simulink model "generic_IVS"  (R2024a)
settings: Solver=FixedStepDiscrete  StartTime=0.0  StopTime=inf  FixedStep=0.001  RelTol=1e-3
undefined symbols (not defined in the file): do_waypoints_tail_shifted_2, pathXY, route1_waypoint, route1_waypoint_raw, route2_waypoint, route2_waypoint_raw, route3_waypoint, route3_waypoint_raw, waypoints2
libraries: CarMaker4SL x431, slpidlib x19, dspsigops x3, simulink x1
(part 3 of 15)

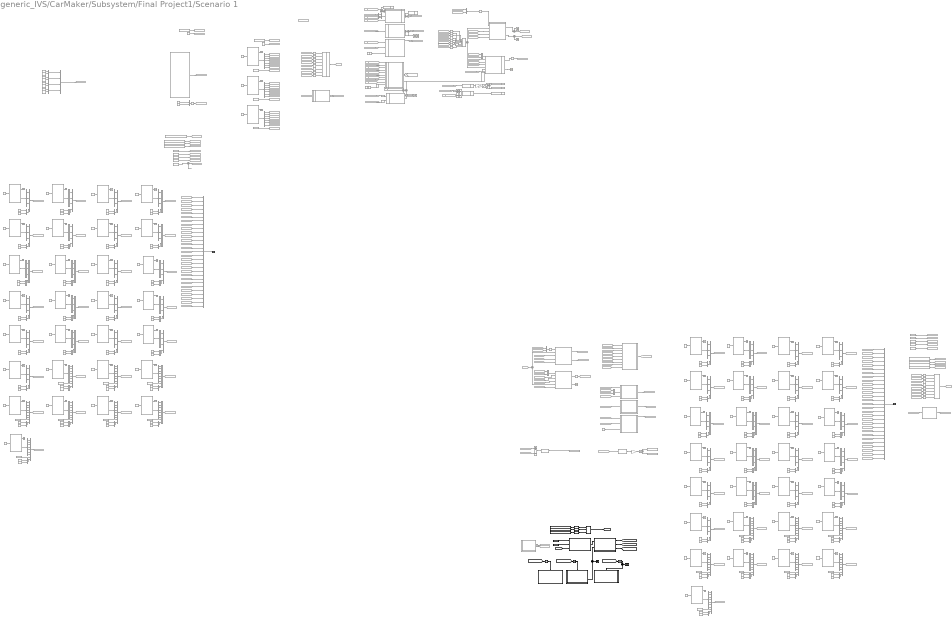
== system generic_IVS/CarMaker/Subsystem/Final Project1/Scenario 1 ==
  note: Average Filter
  note: Do Not Modify !!
  note: Traffic Size
      | Length: 4.47
      | Width: 1.97
      | Height: 1.12
  note: Modify !!
  note: Traffic Size
      | Length: 4.47
      | Width: 1.97
      | Height: 1.12
  note: Traffic Size
      | Length: 4.47
      | Width: 1.97
      | Height: 1.12
  note: *** Final Project ***
      |
      | Scenario:
      | Input:
      | Output:
      | 제어기 10ms / 다익스트라 1s
  note: Do Not Modify !!
  note: Traffic Size
      | Length: 4.47
      | Width: 1.97
      | Height: 1.12
  note: Traffic Size
      | Length: 4.47
      | Width: 1.97
      | Height: 1.12
  note: Traffic Size
      | Length: 4.47
      | Width: 1.97
      | Height: 1.12
  note: Traffic Size
      | Length: 4.47
      | Width: 1.97
      | Height: 1.12
  note: Traffic Size
      | Length: 4.47
      | Width: 1.97
      | Height: 1.12
  note: Traffic Size
      | Length: 4.47
      | Width: 1.97
      | Height: 1.12
  note: Traffic Size
      | Length: 4.47
      | Width: 1.97
      | Height: 1.12
  note: Traffic Size
      | Length: 4.47
      | Width: 1.97
      | Height: 1.12
  note: Traffic Size
      | Length: 4.47
      | Width: 1.97
      | Height: 1.12
  note: Traffic Size
      | Length: 4.47
      | Width: 1.97
      | Height: 1.12
  note: Traffic Size
      | Length: 4.47
      | Width: 1.97
      | Height: 1.12
  note: Traffic Size
      | Length: 4.47
      | Width: 1.97
      | Height: 1.12
  note: Traffic Size
      | Length: 4.47
      | Width: 1.97
      | Height: 1.12
  note: Traffic Size
      | Length: 4.47
      | Width: 1.97
      | Height: 1.12
  note: Traffic Size
      | Length: 4.47
      | Width: 1.97
      | Height: 1.12
  note: Traffic Size
      | Length: 4.47
      | Width: 1.97
      | Height: 1.12
  note: Traffic Size
      | Length: 4.47
      | Width: 1.97
      | Height: 1.12
  note: Traffic Size
      | Length: 4.47
      | Width: 1.97
      | Height: 1.12
  note: Traffic Size
      | Length: 4.47
      | Width: 1.97
      | Height: 1.12
  note: Traffic Size
      | Length: 4.47
      | Width: 1.97
      | Height: 1.12
  note: Traffic Size
      | Length: 4.47
      | Width: 1.97
      | Height: 1.12
  note: Traffic Size
      | Length: 4.47
      | Width: 1.97
      | Height: 1.12
  note: Traffic Size
      | Length: 4.47
      | Width: 1.97
      | Height: 1.12
  note: Traffic Size
      | Length: 4.47
      | Width: 1.97
      | Height: 1.12
  note: Traffic Size
      | Length: 4.47
      | Width: 1.97
      | Height: 1.12
  note: Traffic Size
      | Length: 4.47
      | Width: 1.97
      | Height: 1.12
  note: Traffic Size
      | Length: 4.47
      | Width: 1.97
      | Height: 1.12
  note: Traffic Size
      | Length: 4.47
      | Width: 1.97
      | Height: 1.12
  note: Traffic Size
      | Length: 4.47
      | Width: 1.97
      | Height: 1.12
  note: Traffic Size
      | Length: 4.47
      | Width: 1.97
      | Height: 1.12
  note: Traffic Size
      | Length: 4.47
      | Width: 1.97
      | Height: 1.12
  note: Traffic Size
      | Length: 4.47
      | Width: 1.97
      | Height: 1.12
  note: Traffic Size
      | Length: 4.47
      | Width: 1.97
      | Height: 1.12
  note: *** Final Project ***
      |
      | Scenario:
      | Input:
      | Output:
      | 제어기 10ms / 다익스트라 1s
  note: Traffic Size
      | Length: 4.47
      | Width: 1.97
      | Height: 1.12
  note: Average Filter
  note: Traffic Size
      | Length: 4.47
      | Width: 1.97
      | Height: 1.12
  note: Traffic Size
      | Length: 4.47
      | Width: 1.97
      | Height: 1.12
  note: Traffic Size
      | Length: 4.47
      | Width: 1.97
      | Height: 1.12
  note: Traffic Size
      | Length: 4.47
      | Width: 1.97
      | Height: 1.12
  note: Traffic Size
      | Length: 4.47
      | Width: 1.97
      | Height: 1.12
  note: Traffic Size
      | Length: 4.47
      | Width: 1.97
      | Height: 1.12
  note: Traffic Size
      | Length: 4.47
      | Width: 1.97
      | Height: 1.12
  note: Traffic Size
      | Length: 4.47
      | Width: 1.97
      | Height: 1.12
  note: Traffic Size
      | Length: 4.47
      | Width: 1.97
      | Height: 1.12
  note: Traffic Size
      | Length: 4.47
      | Width: 1.97
      | Height: 1.12
  note: Traffic Size
      | Length: 4.47
      | Width: 1.97
      | Height: 1.12
  note: Traffic Size
      | Length: 4.47
      | Width: 1.97
      | Height: 1.12
  note: Traffic Size
      | Length: 4.47
      | Width: 1.97
      | Height: 1.12
  note: Traffic Size
      | Length: 4.47
      | Width: 1.97
      | Height: 1.12
  note: Traffic Size
      | Length: 4.47
      | Width: 1.97
      | Height: 1.12
  note: Traffic Size
      | Length: 4.47
      | Width: 1.97
      | Height: 1.12
  note: Modify !!
  note: Traffic Size
      | Length: 4.47
      | Width: 1.97
      | Height: 1.12
  note: Traffic Size
      | Length: 4.47
      | Width: 1.97
      | Height: 1.12
  note: Traffic Size
      | Length: 4.47
      | Width: 1.97
      | Height: 1.12
  note: Traffic Size
      | Length: 4.47
      | Width: 1.97
      | Height: 1.12
  note: Traffic Size
      | Length: 4.47
      | Width: 1.97
      | Height: 1.12
  note: Traffic Size
      | Length: 4.47
      | Width: 1.97
      | Height: 1.12
  note: Traffic Size
      | Length: 4.47
      | Width: 1.97
      | Height: 1.12
  note: Traffic Size
      | Length: 4.47
      | Width: 1.97
      | Height: 1.12
  note: Do Not Modify !!
  note: Average Filter
  note: Modify !!
  Add : Sum  Commented=on  Inputs=+-
  Add1 : Sum  Commented=on  Inputs=+-
  Add2 : Sum  Commented=on  Inputs=+-
  Bus Selector{,1..2,20..21,23..27,31,42..43,45..49,54} (19 alike) : BusSelector  Commented=on  OutputSignals=t_0 x,t_0 y,v_0 x,v_0 y,a_0 x,a_0 y,r_zyx z
  Bus Selector{3..19,22,28..30,32..41,44,50..53,55..60} (42 alike) : BusSelector  Commented=on  OutputSignals=t_0 x,t_0 y,r_zyx z
  Chart : Stateflow chart  Commented=on  TreatAsAtomicUnit=on
  Constant : Constant  Commented=on  Value=80
  Constant1 : Constant  Commented=on  Value=0
  Constant10 : Constant  Commented=on  Value=2.48
  Constant100 : Constant  Commented=on  Value=47.5
  Constant101 : Constant  Commented=on  Value=-45
  Constant102 : Constant  Commented=on  Value=5.5
  Constant103 : Constant  Commented=on  Value=-45
  Constant104 : Constant  Commented=on  Value=47.5
  Constant105 : Constant  Commented=on  Value=-4
  Constant106 : Constant  Commented=on  Value=pathXY
  Constant107 : Constant  Commented=on  Value=pathXY
  Constant{2,7,11,108,168,202} (6 alike) : Constant  Commented=on
  Constant109 : Constant  Commented=on  Value=5
  Constant{13,16,19,21..22,26,29,32,35,39,42,46,48,52,55..56,59,61,65,69,72,74,79,82,85,87..88,92,96,110,113,116,118..119,123,126,129,132,136,139,143,145,149,152..153,156,159,163,167,171,173,178,182,185,187..188,193,197} (58 alike) : Constant  Commented=on  Value=4.47
  Constant{14,17,23..24,27,30,33,36..37,40,43,49..50,53,57,62..63,66..67,70,75..76,80,83,89..90,93..94,97,111,114,120..121,124,127,130,133..134,137,140,146..147,150,154,160..161,164..165,169,174..175,180,183,189,191,194..195,198} (58 alike) : Constant  Commented=on  Value=1.97
  Constant112 : Constant  Commented=on  Value=7
  Constant115 : Constant  Commented=on  Value=8
  Constant117 : Constant  Commented=on  Value=4
  Constant12 : Constant  Commented=on  Value=5
  Constant122 : Constant  Commented=on  Value=10
  Constant125 : Constant  Commented=on  Value=11
  Constant128 : Constant  Commented=on  Value=12
  Constant131 : Constant  Commented=on  Value=9
  Constant135 : Constant  Commented=on  Value=14
  Constant138 : Constant  Commented=on  Value=15
  Constant141 : Constant  Commented=on  Value=2
  Constant142 : Constant  Commented=on  Value=16
  Constant144 : Constant  Commented=on  Value=13
  Constant148 : Constant  Commented=on  Value=18
  Constant15 : Constant  Commented=on  Value=7
  Constant151 : Constant  Commented=on  Value=19
  Constant155 : Constant  Commented=on  Value=6
  Constant157 : Constant  Commented=on  Value=route1_waypoint_raw
  Constant158 : Constant  Commented=on  Value=17
  Constant162 : Constant  Commented=on  Value=21
  Constant166 : Constant  Commented=on  Value=22
  Constant170 : Constant  Commented=on  Value=23
  Constant172 : Constant  Commented=on  Value=20
  Constant176 : Constant  Commented=on  Value=3
  Constant177 : Constant  Commented=on  Value=25
  Constant179 : Constant  Commented=on  Value=route2_waypoint_raw
  Constant18 : Constant  Commented=on  Value=8
  Constant181 : Constant  Commented=on  Value=26
  Constant184 : Constant  Commented=on  Value=27
  Constant186 : Constant  Commented=on  Value=24
  Constant190 : Constant  Commented=on  Value=route3_waypoint_raw
  Constant192 : Constant  Commented=on  Value=0
  Constant196 : Constant  Commented=on  Value=28
  Constant199 : Constant  Value=route1_waypoint  SampleTime=-1
  Constant20 : Constant  Commented=on  Value=4
  Constant200 : Constant  Value=route2_waypoint  SampleTime=-1
  Constant201 : Constant  Value=route3_waypoint  SampleTime=-1
  Constant25 : Constant  Commented=on  Value=10
  Constant28 : Constant  Commented=on  Value=11
  Constant3 : Constant  Commented=on  Value=2
  Constant31 : Constant  Commented=on  Value=12
  Constant34 : Constant  Commented=on  Value=9
  Constant38 : Constant  Commented=on  Value=14
  Constant4 : Constant  Commented=on  Value=80
  Constant41 : Constant  Commented=on  Value=15
  Constant44 : Constant  Commented=on  Value=2
  Constant45 : Constant  Commented=on  Value=16
  Constant47 : Constant  Commented=on  Value=13
  Constant5 : Constant  Commented=on  Value=11.5
  Constant51 : Constant  Commented=on  Value=18
  Constant54 : Constant  Commented=on  Value=19
  Constant58 : Constant  Commented=on  Value=6
  Constant6 : Constant  Commented=on  Value=route1_waypoint_raw
  Constant60 : Constant  Commented=on  Value=17
  Constant64 : Constant  Commented=on  Value=21
  Constant68 : Constant  Commented=on  Value=22
  Constant71 : Constant  Commented=on  Value=23
  Constant73 : Constant  Commented=on  Value=20
  Constant77 : Constant  Commented=on  Value=3
  Constant78 : Constant  Commented=on  Value=25
  Constant8 : Constant  Commented=on  Value=route2_waypoint_raw
  Constant81 : Constant  Commented=on  Value=26
  Constant84 : Constant  Commented=on  Value=27
  Constant86 : Constant  Commented=on  Value=24
  Constant9 : Constant  Commented=on  Value=route3_waypoint_raw
  Constant91 : Constant  Commented=on  Value=0
  Constant95 : Constant  Commented=on  Value=28
  Constant98 : Constant  Commented=on  Value=5.5
  Constant99 : Constant  Commented=on  Value=-4
  Display : Display  Commented=on
  Display1 : Display  Commented=on
  Enabled Subsystem : Subsystem  TreatAsAtomicUnit=on
  Enabled Subsystem1 : Subsystem  TreatAsAtomicUnit=on
  Enabled Subsystem2 : Subsystem  TreatAsAtomicUnit=on
  From : From  Commented=on  GotoTag=Traffic_Info_00
  From1 : From  Commented=on  GotoTag=Traffic_Info_01
  From10 : From  Commented=on  GotoTag=Traffic_Info_10
  From100 : From  Commented=on  GotoTag=LateralError
  From101 : From  Commented=on  GotoTag=Global_Waypoints1
  From{2,35,73..74,102,136..137,163} (8 alike) : From  Commented=on  GotoTag=Global_Waypoints2
  From103 : From  Commented=on  GotoTag=Global_Waypoints3
  From{4,28,37,63,77,104,126,133,140,152,155,166} (12 alike) : From  Commented=on  GotoTag=Ego_Global_X
  From{5,29,38,64,78,105,127,141,143,153,156,167} (12 alike) : From  Commented=on  GotoTag=Ego_Gloabl_Y
  From{39,56,69,106,132} (5 alike) : From  Commented=on  GotoTag=Traffic_Info_27
  From107 : From  Commented=on  GotoTag=Traffic_Info_01
  From{40,70,72,108,134} (5 alike) : From  Commented=on  GotoTag=Traffic_Info_28
  From109 : From  Commented=on  GotoTag=Traffic_Info_03
  From11 : From  Commented=on  GotoTag=Traffic_Info_11
  From110 : From  Commented=on  GotoTag=Traffic_Info_04
  From111 : From  Commented=on  GotoTag=Traffic_Info_05
  From112 : From  Commented=on  GotoTag=Traffic_Info_06
  From113 : From  Commented=on  GotoTag=Traffic_Info_07
  From114 : From  Commented=on  GotoTag=Traffic_Info_08
  From115 : From  Commented=on  GotoTag=Traffic_Info_09
  From{76,116,139,165} (4 alike) : From  Commented=on  GotoTag=onRoad_Traffic
  From{8,54,71,79,98,117,135,142,157,168..169} (11 alike) : From  Commented=on  GotoTag=Ego_Velocity
  From{55,82,118,146,158,172} (6 alike) : From  Commented=on  GotoTag=Target_speed2
  From119 : From  Commented=on  GotoTag=Trajectory
  From12 : From  Commented=on  GotoTag=Traffic_Info_12
  From{22,48,58,91,120} (5 alike) : From  Commented=on  GotoTag=Traffic_Info_21
  From{23,49,59,92,121} (5 alike) : From  Commented=on  GotoTag=Traffic_Info_22
  From{3,65,81,122,128,145,154,171} (8 alike) : From  Commented=on  GotoTag=Ego_Yaw
  From{24,50,60,93,123} (5 alike) : From  Commented=on  GotoTag=Traffic_Info_23
  From{25,51,61,94,124} (5 alike) : From  Commented=on  GotoTag=Traffic_Info_24
  From{26,52,62,95,125} (5 alike) : From  Commented=on  GotoTag=Traffic_Info_25
  From129 : From  Commented=on  GotoTag=ego_lane_idx
  From13 : From  Commented=on  GotoTag=Traffic_Info_13
  From130 : From  Commented=on  GotoTag=traffic_lane_idx
  From{27,53,68,96,131} (5 alike) : From  Commented=on  GotoTag=Traffic_Info_26
  From138 : From  Commented=on  GotoTag=s_reference
  From14 : From  Commented=on  GotoTag=Traffic_Info_14
  From144 : From  Commented=on  GotoTag=Ego_Accel
  From147 : From  Commented=on  GotoTag=Local_Points
  From15 : From  Commented=on  GotoTag=Traffic_Info_15
  From159 : From  Commented=on  GotoTag=Trajectory
  From16 : From  Commented=on  GotoTag=Traffic_Info_16
  From160 : From  Commented=on  GotoTag=Local_Points
  From161 : From  Commented=on  GotoTag=traffic_lane_idx
  From162 : From  Commented=on  GotoTag=Coefficients
  From164 : From  Commented=on  GotoTag=s_reference
  From17 : From  Commented=on  GotoTag=Traffic_Info_17
  From170 : From  Commented=on  GotoTag=Ego_Accel
  From173 : From  Commented=on  GotoTag=LateralError
  From18 : From  Commented=on  GotoTag=Traffic_Info_18
  From19 : From  Commented=on  GotoTag=Traffic_Info_19
  From20 : From  Commented=on  GotoTag=Traffic_Info_02
  From21 : From  Commented=on  GotoTag=Traffic_Info_20
  From30 : From  Commented=on  GotoTag=Traffic_Info_10
  From31 : From  Commented=on  GotoTag=Traffic_Info_11
  From32 : From  Commented=on  GotoTag=Traffic_Info_12
  From33 : From  Commented=on  GotoTag=Traffic_Info_13
  From34 : From  Commented=on  GotoTag=Global_Waypoints1
  From36 : From  Commented=on  GotoTag=Global_Waypoints3
  From41 : From  Commented=on  GotoTag=Traffic_Info_03
  From42 : From  Commented=on  GotoTag=Traffic_Info_04
  From43 : From  Commented=on  GotoTag=Traffic_Info_05
  From44 : From  Commented=on  GotoTag=Traffic_Info_06
  From45 : From  Commented=on  GotoTag=Traffic_Info_07
  From46 : From  Commented=on  GotoTag=Traffic_Info_08
  From47 : From  Commented=on  GotoTag=Traffic_Info_09
  From57 : From  Commented=on  GotoTag=Trajectory
  From6 : From  Commented=on  GotoTag=Local_Points
  From66 : From  Commented=on  GotoTag=ego_lane_idx
  From67 : From  Commented=on  GotoTag=traffic_lane_idx
  From7 : From  Commented=on  GotoTag=Coefficients
  From75 : From  Commented=on  GotoTag=s_reference
  From80 : From  Commented=on  GotoTag=Ego_Accel
  From83 : From  Commented=on  GotoTag=Traffic_Info_14
  From84 : From  Commented=on  GotoTag=Traffic_Info_15
  From85 : From  Commented=on  GotoTag=Traffic_Info_16
  From86 : From  Commented=on  GotoTag=Traffic_Info_17
  From87 : From  Commented=on  GotoTag=Traffic_Info_18
  From88 : From  Commented=on  GotoTag=Traffic_Info_19
  From89 : From  Commented=on  GotoTag=Traffic_Info_02
  From9 : From  Commented=on  GotoTag=LateralError
  From90 : From  Commented=on  GotoTag=Traffic_Info_20
  From97 : From  Commented=on  GotoTag=Coefficients
  From99 : From  Commented=on  GotoTag=Traffic_Info_00
  Function-Call Split : FunctionCallSplit  Commented=on  IconShape=distinctive  NumOutputPorts=2  OutputPortLayout=default
  Gain : Gain  Commented=on  Gain=pi/180
  Gain1 : Gain  Commented=on  Gain=pi/180
  Gain2 : Gain  Commented=on  Gain=pi/180
  Goto : Goto  Commented=on  GotoTag=onRoad_Traffic
  Goto1 : Goto  Commented=on  GotoTag=CrossTrackError
  Goto10 : Goto  Commented=on  GotoTag=Traffic00_Yaw
  Goto100 : Goto  Commented=on  GotoTag=Traffic_Info_19
  Goto101 : Goto  Commented=on  GotoTag=Traffic_Info_17
  Goto102 : Goto  Commented=on  GotoTag=Traffic_Info_06
  Goto103 : Goto  Commented=on  GotoTag=Traffic_Info_02
  Goto104 : Goto  Commented=on  GotoTag=Traffic_Info_21
  Goto105 : Goto  Commented=on  GotoTag=Traffic_Info_22
  Goto106 : Goto  Commented=on  GotoTag=Traffic_Info_20
  Goto107 : Goto  Commented=on  GotoTag=Traffic_Info_23
  Goto108 : Goto  Commented=on  GotoTag=Traffic_Info_25
  Goto109 : Goto  Commented=on  GotoTag=Traffic_Info_26
  Goto11 : Goto  Commented=on  GotoTag=Traffic01_Yaw
  Goto110 : Goto  Commented=on  GotoTag=Traffic_Info_24
  Goto111 : Goto  Commented=on  GotoTag=Traffic_Info_27
  Goto112 : Goto  Commented=on  GotoTag=Traffic_Info_00
  Goto113 : Goto  Commented=on  GotoTag=Traffic_Info_03
  Goto114 : Goto  Commented=on  GotoTag=Traffic_Info_28
  Goto115 : Goto  Commented=on  GotoTag=Traffic_Info_05
  Goto116 : Goto  Commented=on  GotoTag=Traffic_Info_07
  Goto117 : Goto  Commented=on  GotoTag=Traffic_Info_04
  Goto118 : Goto  Commented=on  GotoTag=Traffic_Info_08
  Goto119 : Goto  Commented=on  GotoTag=Traffic_Info_10
  Goto12 : Goto  Commented=on  GotoTag=Traffic01_YawRate
  Goto120 : Goto  Commented=on  GotoTag=Traffic_Info_11
  Goto121 : Goto  Commented=on  GotoTag=Global_Waypoints4
  Goto122 : Goto  Commented=on  GotoTag=s_reference
  Goto123 : Goto  Commented=on  GotoTag=Trajectory
  Goto124 : Goto  Commented=on  GotoTag=Ego_Accel
  Goto125 : Goto  Commented=on  GotoTag=do_Logic
  Goto126 : Goto  Commented=on  GotoTag=do_Logic_
  Goto13 : Goto  Commented=on  GotoTag=Traffic01_Global_X
  Goto131 : Goto  Commented=on  GotoTag=Local_Points
  Goto132 : Goto  Commented=on  GotoTag=Coefficients
  Goto133 : Goto  Commented=on  GotoTag=LateralError
  Goto134 : Goto  Commented=on  GotoTag=s_reference
  Goto135 : Goto  Commented=on  GotoTag=Trajectory
  Goto14 : Goto  Commented=on  GotoTag=Traffic01_Global_Y
  Goto15 : Goto  Commented=on  GotoTag=Traffic01_Vx
  Goto16 : Goto  Commented=on  GotoTag=Traffic01_Vy
  Goto17 : Goto  Commented=on  GotoTag=Traffic01_Ax
  Goto18 : Goto  Commented=on  GotoTag=Traffic01_Ay
  Goto19 : Goto  Commented=on  GotoTag=Traffic02_Yaw
  Goto2 : Goto  Commented=on  GotoTag=Traffic00_YawRate
  Goto20 : Goto  Commented=on  GotoTag=Traffic02_YawRate
  Goto21 : Goto  Commented=on  GotoTag=Traffic02_Global_X
  Goto22 : Goto  Commented=on  GotoTag=Traffic02_Global_Y
  Goto23 : Goto  Commented=on  GotoTag=Traffic02_Vx
  Goto24 : Goto  Commented=on  GotoTag=Traffic02_Vy
  Goto25 : Goto  Commented=on  GotoTag=Traffic02_Ax
  Goto26 : Goto  Commented=on  GotoTag=Traffic02_Ay
  Goto27 : Goto  Commented=on  GotoTag=CrossTrackError
  Goto28 : Goto  Commented=on  GotoTag=Traffic_size
  Goto29 : Goto  Commented=on  GotoTag=Target_Speed
  Goto3 : Goto  Commented=on  GotoTag=Traffic00_Global_X
  Goto30 : Goto  Commented=on  GotoTag=Traffic_Info
  Goto31 : Goto  Commented=on  GotoTag=Local_Points
  Goto32 : Goto  Commented=on  GotoTag=Ego_Global_X
  Goto33 : Goto  Commented=on  GotoTag=Ego_Gloabl_Y
  Goto34 : Goto  Commented=on  GotoTag=Ego_Velocity
  Goto35 : Goto  Commented=on  GotoTag=Ego_Yaw
  Goto36 : Goto  Commented=on  GotoTag=Coefficients
  Goto37 : Goto  Commented=on  GotoTag=LateralError
  Goto38 : Goto  Commented=on  GotoTag=Global_Waypoints1
  Goto39 : Goto  Commented=on  GotoTag=Global_Waypoints2
  Goto4 : Goto  Commented=on  GotoTag=Target_Speed
  Goto40 : Goto  Commented=on  GotoTag=Global_Waypoints3
  Goto41 : Goto  Commented=on  GotoTag=Traffic_Info_01
  Goto42 : Goto  Commented=on  GotoTag=traffic_lane_idx
  Goto43 : Goto  Commented=on  GotoTag=ego_lane_idx
  Goto44 : Goto  Commented=on  GotoTag=Traffic_Info_09
  Goto45 : Goto  Commented=on  GotoTag=Target_speed2
  Goto46 : Goto  Commented=on  GotoTag=Traffic_Info_12
  Goto47 : Goto  Commented=on  GotoTag=Traffic_Info_14
  Goto48 : Goto  Commented=on  GotoTag=Traffic_Info_15
  Goto49 : Goto  Commented=on  GotoTag=Traffic_Info_13
  Goto5 : Goto  Commented=on  GotoTag=Traffic00_Global_Y
  Goto50 : Goto  Commented=on  GotoTag=Traffic_Info_16
  Goto51 : Goto  Commented=on  GotoTag=Traffic_Info_18
  Goto52 : Goto  Commented=on  GotoTag=Traffic_Info_19
  Goto53 : Goto  Commented=on  GotoTag=Traffic_Info_17
  Goto54 : Goto  Commented=on  GotoTag=Traffic_Info_06
  Goto55 : Goto  Commented=on  GotoTag=Traffic_Info_02
  Goto56 : Goto  Commented=on  GotoTag=Traffic_Info_21
  Goto57 : Goto  Commented=on  GotoTag=Traffic_Info_22
  Goto58 : Goto  Commented=on  GotoTag=Traffic_Info_20
  Goto59 : Goto  Commented=on  GotoTag=Traffic_Info_23
  Goto6 : Goto  Commented=on  GotoTag=Traffic00_Vx
  Goto60 : Goto  Commented=on  GotoTag=Traffic_Info_25
  Goto61 : Goto  Commented=on  GotoTag=Traffic_Info_26
  Goto62 : Goto  Commented=on  GotoTag=Traffic_Info_24
  Goto63 : Goto  Commented=on  GotoTag=Traffic_Info_27
  Goto64 : Goto  Commented=on  GotoTag=Traffic_Info_00
  Goto65 : Goto  Commented=on  GotoTag=Traffic_Info_03
  Goto66 : Goto  Commented=on  GotoTag=Traffic_Info_28
  Goto67 : Goto  Commented=on  GotoTag=Traffic_Info_05
  Goto68 : Goto  Commented=on  GotoTag=Traffic_Info_07
  Goto69 : Goto  Commented=on  GotoTag=Traffic_Info_04
  Goto7 : Goto  Commented=on  GotoTag=Traffic00_Vy
  Goto70 : Goto  Commented=on  GotoTag=Traffic_Info_08
  Goto71 : Goto  Commented=on  GotoTag=Traffic_Info_10
  Goto72 : Goto  Commented=on  GotoTag=Traffic_Info_11
  Goto73 : Goto  Commented=on  GotoTag=Global_Waypoints4
  Goto74 : Goto  Commented=on  GotoTag=Parking_Map_Boundary
  Goto75 : Goto  Commented=on  GotoTag=Local_Points
  Goto76 : Goto  Commented=on  GotoTag=s_reference
  Goto77 : Goto  Commented=on  GotoTag=Ego_Global_X
  Goto78 : Goto  Commented=on  GotoTag=Trajectory
  Goto79 : Goto  Commented=on  GotoTag=Ego_Accel
  Goto8 : Goto  Commented=on  GotoTag=Traffic00_Ax
  Goto80 : Goto  Commented=on  GotoTag=Ego_Gloabl_Y
  Goto81 : Goto  Commented=on  GotoTag=Ego_Velocity
  Goto82 : Goto  Commented=on  GotoTag=Ego_Yaw
  Goto83 : Goto  Commented=on  GotoTag=Coefficients
  Goto84 : Goto  Commented=on  GotoTag=LateralError
  Goto85 : Goto  Commented=on  GotoTag=Global_Waypoints1
  Goto86 : Goto  Commented=on  GotoTag=Global_Waypoints2
  Goto87 : Goto  Commented=on  GotoTag=Global_Waypoints3
  Goto88 : Goto  Commented=on  GotoTag=Traffic_Info_01
  Goto89 : Goto  Commented=on  GotoTag=traffic_lane_idx
  Goto9 : Goto  Commented=on  GotoTag=Traffic00_Ay
  Goto90 : Goto  Commented=on  GotoTag=ego_lane_idx
  Goto91 : Goto  Commented=on  GotoTag=Traffic_Info_09
  Goto92 : Goto  Commented=on  GotoTag=Target_speed2
  Goto93 : Goto  Commented=on  GotoTag=Traffic_Info_12
  Goto94 : Goto  Commented=on  GotoTag=Traffic_Info_14
  Goto95 : Goto  Commented=on  GotoTag=Traffic_Info_15
  Goto96 : Goto  Commented=on  GotoTag=Traffic_Info_13
  Goto97 : Goto  Commented=on  GotoTag=onRoad_Traffic
  Goto98 : Goto  Commented=on  GotoTag=Traffic_Info_16
  Goto99 : Goto  Commented=on  GotoTag=Traffic_Info_18
  MATLAB Function : MATLAB Function  TreatAsAtomicUnit=on
  MATLAB Function1 : MATLAB Function  Commented=on  TreatAsAtomicUnit=on
  MATLAB Function10 : MATLAB Function  Commented=on  TreatAsAtomicUnit=on
  MATLAB Function11 : MATLAB Function  Commented=on  TreatAsAtomicUnit=on
  MATLAB Function12 : MATLAB Function  Commented=on  TreatAsAtomicUnit=on
  MATLAB Function13 : MATLAB Function  Commented=on  TreatAsAtomicUnit=on
  MATLAB Function14 : MATLAB Function  TreatAsAtomicUnit=on
  MATLAB Function15 : MATLAB Function  Commented=on  TreatAsAtomicUnit=on
  MATLAB Function16 : MATLAB Function  Commented=on  TreatAsAtomicUnit=on
  MATLAB Function17 : MATLAB Function  Commented=on  TreatAsAtomicUnit=on
  MATLAB Function18 : MATLAB Function  Commented=on  TreatAsAtomicUnit=on
  MATLAB Function19 : MATLAB Function  Commented=on  TreatAsAtomicUnit=on
  MATLAB Function2 : MATLAB Function  Commented=on  TreatAsAtomicUnit=on
  MATLAB Function20 : MATLAB Function  Commented=on  TreatAsAtomicUnit=on
  MATLAB Function3 : MATLAB Function  Commented=on  TreatAsAtomicUnit=on
  MATLAB Function4 : MATLAB Function  Commented=on  TreatAsAtomicUnit=on
  "MATLAB Function4 " : MATLAB Function  Commented=on  TreatAsAtomicUnit=on
  MATLAB Function4 1 : MATLAB Function  Commented=on  TreatAsAtomicUnit=on
  MATLAB Function4 2 : MATLAB Function  Commented=on  TreatAsAtomicUnit=on
  MATLAB Function5 : MATLAB Function  Commented=on  TreatAsAtomicUnit=on
  MATLAB Function6 : MATLAB Function  Commented=on  TreatAsAtomicUnit=on
  MATLAB Function7 : MATLAB Function  Commented=on  TreatAsAtomicUnit=on
  MATLAB Function8 : MATLAB Function  Commented=on  TreatAsAtomicUnit=on
  MATLAB Function9 : MATLAB Function  Commented=on  TreatAsAtomicUnit=on
  Matrix Concatenate{,1..2,4} (4 alike) : Concatenate  Commented=on  NumInputs=8  Mode=Multidimensional array
  Matrix Concatenate3 : Concatenate  NumInputs=3  Mode=Multidimensional array
  Mux{,2..4,6..8,11,13,15,17,19,21,23,25,27,29,31,33,35,37,39,41,43,45,47,49,51,53,55..56,58,61,63,65,67..69,71,73,75,77,79..80,82,84,86,88,90,92,94,96,98,100..101,103,105,107,109,111,114,116,118..119,121,123,125,127..128,130} (70 alike) : Mux  Commented=on  Inputs=2
  Mux{1,5,9..10,12,14,16,18,20,22,24,26,28,30,32,34,36,38,46,57,60,62,66,70,72,74,76,78,81,83,85,87,89,91,93,95,97,99,108,112,120,124,129} (43 alike) : Mux  Commented=on
  Mux{40,42,44,48,50,52,54,64,102,104,106,110,113,115,117,126} (16 alike) : Mux  Commented=on  Inputs=9
  Mux122 : Mux  Commented=on  Inputs=29
  Mux59 : Mux  Commented=on  Inputs=29
  PID Controller : slpidlib/PID Controller  Commented=on  Controller=PID  Form=Ideal  TimeDomain=Discrete-time  UseExternalTs=off  SampleTime=-1  IntegratorMethod=Forward Euler  FilterMethod=Forward Euler  ControllerParametersSource=internal  P=2  I=0.001  UseKiTs=off  D=0.1  UseExternalDerivativeSource=off  N=1000  UseFilter=off  TunerSelectOption=Transfer Function Based (PID Tuner App)  InitialConditionSource=internal  InitialConditionForIntegrator=0  InitialConditionForFilter=0  DifferentiatorICPrevScaledInput=0  ExternalReset=none  TrackingMode=off  Kt=1  LimitOutput=off  SatLimitsSource=internal  UpperSaturationLimit=1  LowerSaturationLimit=-1  LinearizeAsGain=on  AntiWindupMode=back-calculation  Kb=1  LimitIntegrator=on  UpperIntegratorSaturationLimit=0.7  LowerIntegratorSaturationLimit=-0.7  POutMin=[]  POutMax=[]  IOutMin=[]  IOutMax=[]  DOutMin=[]  DOutMax=[]  NOutMin=[]  NOutMax=[]  SumOutMin=[]  SumOutMax=[]  SaturationOutMin=[]  SaturationOutMax=[]  PParamMin=[]  PParamMax=[]  IParamMin=[]  IParamMax=[]  DParamMin=[]  DParamMax=[]  NParamMin=[]  NParamMax=[]  KbParamMin=[]  KbParamMax=[]  KtParamMin=[]  KtParamMax=[]  KbOutMin=[]  KbOutMax=[]  KtOutMin=[]  KtOutMax=[]  IntegratorOutMin=[]  IntegratorOutMax=[]  FilterOutMin=[]  FilterOutMax=[]  SumI1OutMin=[]  SumI1OutMax=[]  SumI2OutMin=[]  SumI2OutMax=[]  SumI3OutMin=[]  SumI3OutMax=[]  SumI4OutMin=[]  SumI4OutMax=[]  SumDOutMin=[]  SumDOutMax=[]  DifferentiatorOutMin=[]  DifferentiatorOutMax=[]  FilterDiffOutCoefMin=[]  FilterDiffOutCoefMax=[]  ReciprocalOutMin=[]  ReciprocalOutMax=[]  SumDenOutMin=[]  SumDenOutMax=[]  SumNumOutMin=[]  SumNumOutMax=[]  DivideOutMin=[]  DivideOutMax=[]  UdiffTsProdOutMin=[]  UdiffTsProdOutMax=[]  NTsProdOutMin=[]  NTsProdOutMax=[]  UintegralTsProdOutMin=[]  UintegralTsProdOutMax=[]  UngainTsProdOutMin=[]  UngainTsProdOutMax=[]  ClampingZeroOutDataTypeStr=Inherit: Inherit via back propagation  ClampingZeroOutMin=[]  ClampingZeroOutMax=[]  FilterDenConstantOutDataTypeStr=Inherit: Inherit via back propagation  FilterDenConstantOutMin=[]  FilterDenConstantOutMax=[]  PCopyOutDataTypeStr=Inherit: Inherit via back propagation  PCopyOutMin=[]  PCopyOutMax=[]  NCopyOutDataTypeStr=Inherit: Inherit via back propagation  NCopyOutMin=[]  NCopyOutMax=[]  IntegratorContinuousStateAttributes=''  IntegratorStateMustResolveToSignalObject=off  IntegratorRTWStateStorageClass=Auto  FilterContinuousStateAttributes=''  FilterStateMustResolveToSignalObject=off  FilterRTWStateStorageClass=Auto  ParallelPVariant=Passthrough  IdealPVariant=InternalParameters  IVariant=InternalParameters  DVariant=InternalParameters  IntegratorVariant=Discrete  SatVariant=Disabled  AWVariant=Passthrough  PCopyVariant=Disabled  TRVariant=Disabled  FdbkBlocksVariant=Forward  IdealPFdbkVariant=Disabled  SatFdbkVariant=Disabled  DerivativeFilterVariant=Differentiator  NVariant=Passthrough  NCopyVariant=Disabled_SignalSpec  FilterICVariant=InternalICsDifferentiator  IntegratorICVariant=InternalICs  ExternalResetVariant=Disabled  TRSumVariant=Passthrough  SumFdbkVariant=Disabled  SumVariant=Sum_PID  TsampFilterVariant=InternalTs  TsampNgainVariant=Passthrough  TsampIntegralVariant=Disabled_SignalSpec  ExternalSaturationOutDataTypeStr=Inherit: Same as second input  DerivativeSourceVariant=ErrorSignal
  PID Controller1 : slpidlib/PID Controller  Commented=on  Controller=PID  Form=Ideal  TimeDomain=Discrete-time  UseExternalTs=off  SampleTime=-1  IntegratorMethod=Forward Euler  FilterMethod=Forward Euler  ControllerParametersSource=internal  P=3.2  I=0  UseKiTs=off  D=1  UseExternalDerivativeSource=off  N=1000  UseFilter=off  TunerSelectOption=Transfer Function Based (PID Tuner App)  InitialConditionSource=internal  InitialConditionForIntegrator=0  InitialConditionForFilter=0  DifferentiatorICPrevScaledInput=0  ExternalReset=none  TrackingMode=off  Kt=1  LimitOutput=off  SatLimitsSource=internal  UpperSaturationLimit=1  LowerSaturationLimit=-1  LinearizeAsGain=on  AntiWindupMode=back-calculation  Kb=1  LimitIntegrator=off  UpperIntegratorSaturationLimit=0.7  LowerIntegratorSaturationLimit=-0.7  POutMin=[]  POutMax=[]  IOutMin=[]  IOutMax=[]  DOutMin=[]  DOutMax=[]  NOutMin=[]  NOutMax=[]  SumOutMin=[]  SumOutMax=[]  SaturationOutMin=[]  SaturationOutMax=[]  PParamMin=[]  PParamMax=[]  IParamMin=[]  IParamMax=[]  DParamMin=[]  DParamMax=[]  NParamMin=[]  NParamMax=[]  KbParamMin=[]  KbParamMax=[]  KtParamMin=[]  KtParamMax=[]  KbOutMin=[]  KbOutMax=[]  KtOutMin=[]  KtOutMax=[]  IntegratorOutMin=[]  IntegratorOutMax=[]  FilterOutMin=[]  FilterOutMax=[]  SumI1OutMin=[]  SumI1OutMax=[]  SumI2OutMin=[]  SumI2OutMax=[]  SumI3OutMin=[]  SumI3OutMax=[]  SumI4OutMin=[]  SumI4OutMax=[]  SumDOutMin=[]  SumDOutMax=[]  DifferentiatorOutMin=[]  DifferentiatorOutMax=[]  FilterDiffOutCoefMin=[]  FilterDiffOutCoefMax=[]  ReciprocalOutMin=[]  ReciprocalOutMax=[]  SumDenOutMin=[]  SumDenOutMax=[]  SumNumOutMin=[]  SumNumOutMax=[]  DivideOutMin=[]  DivideOutMax=[]  UdiffTsProdOutMin=[]  UdiffTsProdOutMax=[]  NTsProdOutMin=[]  NTsProdOutMax=[]  UintegralTsProdOutMin=[]  UintegralTsProdOutMax=[]  UngainTsProdOutMin=[]  UngainTsProdOutMax=[]  ClampingZeroOutDataTypeStr=Inherit: Inherit via back propagation  ClampingZeroOutMin=[]  ClampingZeroOutMax=[]  FilterDenConstantOutDataTypeStr=Inherit: Inherit via back propagation  FilterDenConstantOutMin=[]  FilterDenConstantOutMax=[]  PCopyOutDataTypeStr=Inherit: Inherit via back propagation  PCopyOutMin=[]  PCopyOutMax=[]  NCopyOutDataTypeStr=Inherit: Inherit via back propagation  NCopyOutMin=[]  NCopyOutMax=[]  IntegratorContinuousStateAttributes=''  IntegratorStateMustResolveToSignalObject=off  IntegratorRTWStateStorageClass=Auto  FilterContinuousStateAttributes=''  FilterStateMustResolveToSignalObject=off  FilterRTWStateStorageClass=Auto  ParallelPVariant=Passthrough  IdealPVariant=InternalParameters  IVariant=InternalParameters  DVariant=InternalParameters  IntegratorVariant=Discrete  SatVariant=Disabled  AWVariant=Passthrough  PCopyVariant=Disabled  TRVariant=Disabled  FdbkBlocksVariant=Forward  IdealPFdbkVariant=Disabled  SatFdbkVariant=Disabled  DerivativeFilterVariant=Differentiator  NVariant=Passthrough  NCopyVariant=Disabled_SignalSpec  FilterICVariant=InternalICsDifferentiator  IntegratorICVariant=InternalICs  ExternalResetVariant=Disabled  TRSumVariant=Passthrough  SumFdbkVariant=Disabled  SumVariant=Sum_PID  TsampFilterVariant=InternalTs  TsampNgainVariant=Passthrough  TsampIntegralVariant=Disabled_SignalSpec  ExternalSaturationOutDataTypeStr=Inherit: Same as second input  DerivativeSourceVariant=ErrorSignal
  PID Controller2 : slpidlib/PID Controller  Commented=on  Controller=PID  Form=Ideal  TimeDomain=Discrete-time  UseExternalTs=off  SampleTime=-1  IntegratorMethod=Forward Euler  FilterMethod=Forward Euler  ControllerParametersSource=internal  P=2  I=0  UseKiTs=off  D=0.2  UseExternalDerivativeSource=off  N=1000  UseFilter=off  TunerSelectOption=Transfer Function Based (PID Tuner App)  InitialConditionSource=internal  InitialConditionForIntegrator=0  InitialConditionForFilter=0  DifferentiatorICPrevScaledInput=0  ExternalReset=none  TrackingMode=off  Kt=1  LimitOutput=off  SatLimitsSource=internal  UpperSaturationLimit=1  LowerSaturationLimit=-1  LinearizeAsGain=on  AntiWindupMode=back-calculation  Kb=1  LimitIntegrator=off  UpperIntegratorSaturationLimit=0.7  LowerIntegratorSaturationLimit=-0.7  POutMin=[]  POutMax=[]  IOutMin=[]  IOutMax=[]  DOutMin=[]  DOutMax=[]  NOutMin=[]  NOutMax=[]  SumOutMin=[]  SumOutMax=[]  SaturationOutMin=[]  SaturationOutMax=[]  PParamMin=[]  PParamMax=[]  IParamMin=[]  IParamMax=[]  DParamMin=[]  DParamMax=[]  NParamMin=[]  NParamMax=[]  KbParamMin=[]  KbParamMax=[]  KtParamMin=[]  KtParamMax=[]  KbOutMin=[]  KbOutMax=[]  KtOutMin=[]  KtOutMax=[]  IntegratorOutMin=[]  IntegratorOutMax=[]  FilterOutMin=[]  FilterOutMax=[]  SumI1OutMin=[]  SumI1OutMax=[]  SumI2OutMin=[]  SumI2OutMax=[]  SumI3OutMin=[]  SumI3OutMax=[]  SumI4OutMin=[]  SumI4OutMax=[]  SumDOutMin=[]  SumDOutMax=[]  DifferentiatorOutMin=[]  DifferentiatorOutMax=[]  FilterDiffOutCoefMin=[]  FilterDiffOutCoefMax=[]  ReciprocalOutMin=[]  ReciprocalOutMax=[]  SumDenOutMin=[]  SumDenOutMax=[]  SumNumOutMin=[]  SumNumOutMax=[]  DivideOutMin=[]  DivideOutMax=[]  UdiffTsProdOutMin=[]  UdiffTsProdOutMax=[]  NTsProdOutMin=[]  NTsProdOutMax=[]  UintegralTsProdOutMin=[]  UintegralTsProdOutMax=[]  UngainTsProdOutMin=[]  UngainTsProdOutMax=[]  ClampingZeroOutDataTypeStr=Inherit: Inherit via back propagation  ClampingZeroOutMin=[]  ClampingZeroOutMax=[]  FilterDenConstantOutDataTypeStr=Inherit: Inherit via back propagation  FilterDenConstantOutMin=[]  FilterDenConstantOutMax=[]  PCopyOutDataTypeStr=Inherit: Inherit via back propagation  PCopyOutMin=[]  PCopyOutMax=[]  NCopyOutDataTypeStr=Inherit: Inherit via back propagation  NCopyOutMin=[]  NCopyOutMax=[]  IntegratorContinuousStateAttributes=''  IntegratorStateMustResolveToSignalObject=off  IntegratorRTWStateStorageClass=Auto  FilterContinuousStateAttributes=''  FilterStateMustResolveToSignalObject=off  FilterRTWStateStorageClass=Auto  ParallelPVariant=Passthrough  IdealPVariant=InternalParameters  IVariant=InternalParameters  DVariant=InternalParameters  IntegratorVariant=Discrete  SatVariant=Disabled  AWVariant=Passthrough  PCopyVariant=Disabled  TRVariant=Disabled  FdbkBlocksVariant=Forward  IdealPFdbkVariant=Disabled  SatFdbkVariant=Disabled  DerivativeFilterVariant=Differentiator  NVariant=Passthrough  NCopyVariant=Disabled_SignalSpec  FilterICVariant=InternalICsDifferentiator  IntegratorICVariant=InternalICs  ExternalResetVariant=Disabled  TRSumVariant=Passthrough  SumFdbkVariant=Disabled  SumVariant=Sum_PID  TsampFilterVariant=InternalTs  TsampNgainVariant=Passthrough  TsampIntegralVariant=Disabled_SignalSpec  ExternalSaturationOutDataTypeStr=Inherit: Same as second input  DerivativeSourceVariant=ErrorSignal
  PID Controller3 : slpidlib/PID Controller  Commented=on  Controller=PID  Form=Ideal  TimeDomain=Discrete-time  UseExternalTs=off  SampleTime=-1  IntegratorMethod=Forward Euler  FilterMethod=Forward Euler  ControllerParametersSource=internal  P=3.2  I=0  UseKiTs=off  D=1  UseExternalDerivativeSource=off  N=1000  UseFilter=off  TunerSelectOption=Transfer Function Based (PID Tuner App)  InitialConditionSource=internal  InitialConditionForIntegrator=0  InitialConditionForFilter=0  DifferentiatorICPrevScaledInput=0  ExternalReset=none  TrackingMode=off  Kt=1  LimitOutput=off  SatLimitsSource=internal  UpperSaturationLimit=1  LowerSaturationLimit=-1  LinearizeAsGain=on  AntiWindupMode=back-calculation  Kb=1  LimitIntegrator=off  UpperIntegratorSaturationLimit=0.7  LowerIntegratorSaturationLimit=-0.7  POutMin=[]  POutMax=[]  IOutMin=[]  IOutMax=[]  DOutMin=[]  DOutMax=[]  NOutMin=[]  NOutMax=[]  SumOutMin=[]  SumOutMax=[]  SaturationOutMin=[]  SaturationOutMax=[]  PParamMin=[]  PParamMax=[]  IParamMin=[]  IParamMax=[]  DParamMin=[]  DParamMax=[]  NParamMin=[]  NParamMax=[]  KbParamMin=[]  KbParamMax=[]  KtParamMin=[]  KtParamMax=[]  KbOutMin=[]  KbOutMax=[]  KtOutMin=[]  KtOutMax=[]  IntegratorOutMin=[]  IntegratorOutMax=[]  FilterOutMin=[]  FilterOutMax=[]  SumI1OutMin=[]  SumI1OutMax=[]  SumI2OutMin=[]  SumI2OutMax=[]  SumI3OutMin=[]  SumI3OutMax=[]  SumI4OutMin=[]  SumI4OutMax=[]  SumDOutMin=[]  SumDOutMax=[]  DifferentiatorOutMin=[]  DifferentiatorOutMax=[]  FilterDiffOutCoefMin=[]  FilterDiffOutCoefMax=[]  ReciprocalOutMin=[]  ReciprocalOutMax=[]  SumDenOutMin=[]  SumDenOutMax=[]  SumNumOutMin=[]  SumNumOutMax=[]  DivideOutMin=[]  DivideOutMax=[]  UdiffTsProdOutMin=[]  UdiffTsProdOutMax=[]  NTsProdOutMin=[]  NTsProdOutMax=[]  UintegralTsProdOutMin=[]  UintegralTsProdOutMax=[]  UngainTsProdOutMin=[]  UngainTsProdOutMax=[]  ClampingZeroOutDataTypeStr=Inherit: Inherit via back propagation  ClampingZeroOutMin=[]  ClampingZeroOutMax=[]  FilterDenConstantOutDataTypeStr=Inherit: Inherit via back propagation  FilterDenConstantOutMin=[]  FilterDenConstantOutMax=[]  PCopyOutDataTypeStr=Inherit: Inherit via back propagation  PCopyOutMin=[]  PCopyOutMax=[]  NCopyOutDataTypeStr=Inherit: Inherit via back propagation  NCopyOutMin=[]  NCopyOutMax=[]  IntegratorContinuousStateAttributes=''  IntegratorStateMustResolveToSignalObject=off  IntegratorRTWStateStorageClass=Auto  FilterContinuousStateAttributes=''  FilterStateMustResolveToSignalObject=off  FilterRTWStateStorageClass=Auto  ParallelPVariant=Passthrough  IdealPVariant=InternalParameters  IVariant=InternalParameters  DVariant=InternalParameters  IntegratorVariant=Discrete  SatVariant=Disabled  AWVariant=Passthrough  PCopyVariant=Disabled  TRVariant=Disabled  FdbkBlocksVariant=Forward  IdealPFdbkVariant=Disabled  SatFdbkVariant=Disabled  DerivativeFilterVariant=Differentiator  NVariant=Passthrough  NCopyVariant=Disabled_SignalSpec  FilterICVariant=InternalICsDifferentiator  IntegratorICVariant=InternalICs  ExternalResetVariant=Disabled  TRSumVariant=Passthrough  SumFdbkVariant=Disabled  SumVariant=Sum_PID  TsampFilterVariant=InternalTs  TsampNgainVariant=Passthrough  TsampIntegralVariant=Disabled_SignalSpec  ExternalSaturationOutDataTypeStr=Inherit: Same as second input  DerivativeSourceVariant=ErrorSignal
  PID Controller4 : slpidlib/PID Controller  Commented=on  Controller=PID  Form=Ideal  TimeDomain=Discrete-time  UseExternalTs=off  SampleTime=-1  IntegratorMethod=Forward Euler  FilterMethod=Forward Euler  ControllerParametersSource=internal  P=2  I=0.001  UseKiTs=off  D=0.1  UseExternalDerivativeSource=off  N=1000  UseFilter=off  TunerSelectOption=Transfer Function Based (PID Tuner App)  InitialConditionSource=internal  InitialConditionForIntegrator=0  InitialConditionForFilter=0  DifferentiatorICPrevScaledInput=0  ExternalReset=none  TrackingMode=off  Kt=1  LimitOutput=off  SatLimitsSource=internal  UpperSaturationLimit=1  LowerSaturationLimit=-1  LinearizeAsGain=on  AntiWindupMode=back-calculation  Kb=1  LimitIntegrator=on  UpperIntegratorSaturationLimit=0.7  LowerIntegratorSaturationLimit=-0.7  POutMin=[]  POutMax=[]  IOutMin=[]  IOutMax=[]  DOutMin=[]  DOutMax=[]  NOutMin=[]  NOutMax=[]  SumOutMin=[]  SumOutMax=[]  SaturationOutMin=[]  SaturationOutMax=[]  PParamMin=[]  PParamMax=[]  IParamMin=[]  IParamMax=[]  DParamMin=[]  DParamMax=[]  NParamMin=[]  NParamMax=[]  KbParamMin=[]  KbParamMax=[]  KtParamMin=[]  KtParamMax=[]  KbOutMin=[]  KbOutMax=[]  KtOutMin=[]  KtOutMax=[]  IntegratorOutMin=[]  IntegratorOutMax=[]  FilterOutMin=[]  FilterOutMax=[]  SumI1OutMin=[]  SumI1OutMax=[]  SumI2OutMin=[]  SumI2OutMax=[]  SumI3OutMin=[]  SumI3OutMax=[]  SumI4OutMin=[]  SumI4OutMax=[]  SumDOutMin=[]  SumDOutMax=[]  DifferentiatorOutMin=[]  DifferentiatorOutMax=[]  FilterDiffOutCoefMin=[]  FilterDiffOutCoefMax=[]  ReciprocalOutMin=[]  ReciprocalOutMax=[]  SumDenOutMin=[]  SumDenOutMax=[]  SumNumOutMin=[]  SumNumOutMax=[]  DivideOutMin=[]  DivideOutMax=[]  UdiffTsProdOutMin=[]  UdiffTsProdOutMax=[]  NTsProdOutMin=[]  NTsProdOutMax=[]  UintegralTsProdOutMin=[]  UintegralTsProdOutMax=[]  UngainTsProdOutMin=[]  UngainTsProdOutMax=[]  ClampingZeroOutDataTypeStr=Inherit: Inherit via back propagation  ClampingZeroOutMin=[]  ClampingZeroOutMax=[]  FilterDenConstantOutDataTypeStr=Inherit: Inherit via back propagation  FilterDenConstantOutMin=[]  FilterDenConstantOutMax=[]  PCopyOutDataTypeStr=Inherit: Inherit via back propagation  PCopyOutMin=[]  PCopyOutMax=[]  NCopyOutDataTypeStr=Inherit: Inherit via back propagation  NCopyOutMin=[]  NCopyOutMax=[]  IntegratorContinuousStateAttributes=''  IntegratorStateMustResolveToSignalObject=off  IntegratorRTWStateStorageClass=Auto  FilterContinuousStateAttributes=''  FilterStateMustResolveToSignalObject=off  FilterRTWStateStorageClass=Auto  ParallelPVariant=Passthrough  IdealPVariant=InternalParameters  IVariant=InternalParameters  DVariant=InternalParameters  IntegratorVariant=Discrete  SatVariant=Disabled  AWVariant=Passthrough  PCopyVariant=Disabled  TRVariant=Disabled  FdbkBlocksVariant=Forward  IdealPFdbkVariant=Disabled  SatFdbkVariant=Disabled  DerivativeFilterVariant=Differentiator  NVariant=Passthrough  NCopyVariant=Disabled_SignalSpec  FilterICVariant=InternalICsDifferentiator  IntegratorICVariant=InternalICs  ExternalResetVariant=Disabled  TRSumVariant=Passthrough  SumFdbkVariant=Disabled  SumVariant=Sum_PID  TsampFilterVariant=InternalTs  TsampNgainVariant=Passthrough  TsampIntegralVariant=Disabled_SignalSpec  ExternalSaturationOutDataTypeStr=Inherit: Same as second input  DerivativeSourceVariant=ErrorSignal
  PID Controller5 : slpidlib/PID Controller  Commented=on  Controller=PID  Form=Ideal  TimeDomain=Discrete-time  UseExternalTs=off  SampleTime=-1  IntegratorMethod=Forward Euler  FilterMethod=Forward Euler  ControllerParametersSource=internal  P=3.2  I=0  UseKiTs=off  D=1  UseExternalDerivativeSource=off  N=1000  UseFilter=off  TunerSelectOption=Transfer Function Based (PID Tuner App)  InitialConditionSource=internal  InitialConditionForIntegrator=0  InitialConditionForFilter=0  DifferentiatorICPrevScaledInput=0  ExternalReset=none  TrackingMode=off  Kt=1  LimitOutput=off  SatLimitsSource=internal  UpperSaturationLimit=1  LowerSaturationLimit=-1  LinearizeAsGain=on  AntiWindupMode=back-calculation  Kb=1  LimitIntegrator=off  UpperIntegratorSaturationLimit=0.7  LowerIntegratorSaturationLimit=-0.7  POutMin=[]  POutMax=[]  IOutMin=[]  IOutMax=[]  DOutMin=[]  DOutMax=[]  NOutMin=[]  NOutMax=[]  SumOutMin=[]  SumOutMax=[]  SaturationOutMin=[]  SaturationOutMax=[]  PParamMin=[]  PParamMax=[]  IParamMin=[]  IParamMax=[]  DParamMin=[]  DParamMax=[]  NParamMin=[]  NParamMax=[]  KbParamMin=[]  KbParamMax=[]  KtParamMin=[]  KtParamMax=[]  KbOutMin=[]  KbOutMax=[]  KtOutMin=[]  KtOutMax=[]  IntegratorOutMin=[]  IntegratorOutMax=[]  FilterOutMin=[]  FilterOutMax=[]  SumI1OutMin=[]  SumI1OutMax=[]  SumI2OutMin=[]  SumI2OutMax=[]  SumI3OutMin=[]  SumI3OutMax=[]  SumI4OutMin=[]  SumI4OutMax=[]  SumDOutMin=[]  SumDOutMax=[]  DifferentiatorOutMin=[]  DifferentiatorOutMax=[]  FilterDiffOutCoefMin=[]  FilterDiffOutCoefMax=[]  ReciprocalOutMin=[]  ReciprocalOutMax=[]  SumDenOutMin=[]  SumDenOutMax=[]  SumNumOutMin=[]  SumNumOutMax=[]  DivideOutMin=[]  DivideOutMax=[]  UdiffTsProdOutMin=[]  UdiffTsProdOutMax=[]  NTsProdOutMin=[]  NTsProdOutMax=[]  UintegralTsProdOutMin=[]  UintegralTsProdOutMax=[]  UngainTsProdOutMin=[]  UngainTsProdOutMax=[]  ClampingZeroOutDataTypeStr=Inherit: Inherit via back propagation  ClampingZeroOutMin=[]  ClampingZeroOutMax=[]  FilterDenConstantOutDataTypeStr=Inherit: Inherit via back propagation  FilterDenConstantOutMin=[]  FilterDenConstantOutMax=[]  PCopyOutDataTypeStr=Inherit: Inherit via back propagation  PCopyOutMin=[]  PCopyOutMax=[]  NCopyOutDataTypeStr=Inherit: Inherit via back propagation  NCopyOutMin=[]  NCopyOutMax=[]  IntegratorContinuousStateAttributes=''  IntegratorStateMustResolveToSignalObject=off  IntegratorRTWStateStorageClass=Auto  FilterContinuousStateAttributes=''  FilterStateMustResolveToSignalObject=off  FilterRTWStateStorageClass=Auto  ParallelPVariant=Passthrough  IdealPVariant=InternalParameters  IVariant=InternalParameters  DVariant=InternalParameters  IntegratorVariant=Discrete  SatVariant=Disabled  AWVariant=Passthrough  PCopyVariant=Disabled  TRVariant=Disabled  FdbkBlocksVariant=Forward  IdealPFdbkVariant=Disabled  SatFdbkVariant=Disabled  DerivativeFilterVariant=Differentiator  NVariant=Passthrough  NCopyVariant=Disabled_SignalSpec  FilterICVariant=InternalICsDifferentiator  IntegratorICVariant=InternalICs  ExternalResetVariant=Disabled  TRSumVariant=Passthrough  SumFdbkVariant=Disabled  SumVariant=Sum_PID  TsampFilterVariant=InternalTs  TsampNgainVariant=Passthrough  TsampIntegralVariant=Disabled_SignalSpec  ExternalSaturationOutDataTypeStr=Inherit: Same as second input  DerivativeSourceVariant=ErrorSignal
  Pad : dspsigops/Pad  padAlong=Columns and rows  dimsToPad=1  valSrc=Specify via dialog  padVal=0  spec=Output size  padNumOutRowsSpecMethod=User-specified  numOutRows=240  padNumOutColsSpecMethod=User-specified  numOutCols=2  isVarDimsMode=off  padBeginning=0  padEnd=0  outSizeMode=User-specified  outSize=1  padSigAt=End  trunc_flag=None  roundingMode=Floor  overflowMode=off  truncOrWrapMode=Truncate  wrap_flag=None
  Pad1 : dspsigops/Pad  padAlong=Columns and rows  dimsToPad=1  valSrc=Specify via dialog  padVal=0  spec=Output size  padNumOutRowsSpecMethod=User-specified  numOutRows=240  padNumOutColsSpecMethod=User-specified  numOutCols=2  isVarDimsMode=off  padBeginning=0  padEnd=0  outSizeMode=User-specified  outSize=1  padSigAt=End  trunc_flag=None  roundingMode=Floor  overflowMode=off  truncOrWrapMode=Truncate  wrap_flag=None
  Pad2 : dspsigops/Pad  padAlong=Columns and rows  dimsToPad=1  valSrc=Specify via dialog  padVal=0  spec=Output size  padNumOutRowsSpecMethod=User-specified  numOutRows=240  padNumOutColsSpecMethod=User-specified  numOutCols=2  isVarDimsMode=off  padBeginning=0  padEnd=0  outSizeMode=User-specified  outSize=1  padSigAt=End  trunc_flag=None  roundingMode=Floor  overflowMode=off  truncOrWrapMode=Truncate  wrap_flag=None
  Rate Limiter : RateLimiter  Commented=on  FallingSlewLimit=-3.0  SampleTimeMode=inherited  InitialCondition=13.0
  Rate Limiter1 : RateLimiter  Commented=on  RisingSlewLimit=1.0  FallingSlewLimit=-3.0  SampleTimeMode=inherited  InitialCondition=13.0
  Read CM Dict : CarMaker4SL/Read CM Dict  Commented=on  xname=Car.Road.Path.DevDist  xsync=off  xstime=Inherited
  Read CM Dict1 : CarMaker4SL/Read CM Dict  Commented=on  xname=Traffic.T22.rzv  xsync=off  xstime=Inherited
  Read CM Dict10 : CarMaker4SL/Read CM Dict  Commented=on  xname=Traffic.T21.rzv  xsync=off  xstime=Inherited
  Read CM Dict11 : CarMaker4SL/Read CM Dict  Commented=on  xname=Traffic.T22.rzv  xsync=off  xstime=Inherited
  Read CM Dict12 : CarMaker4SL/Read CM Dict  Commented=on  xname=Traffic.T23.rzv  xsync=off  xstime=Inherited
  Read CM Dict13 : CarMaker4SL/Read CM Dict  Commented=on  xname=Traffic.T24.rzv  xsync=off  xstime=Inherited
  Read CM Dict14 : CarMaker4SL/Read CM Dict  Commented=on  xname=Traffic.T25.rzv  xsync=off  xstime=Inherited
  Read CM Dict15 : CarMaker4SL/Read CM Dict  Commented=on  xname=Traffic.T26.rzv  xsync=off  xstime=Inherited
  Read CM Dict16 : CarMaker4SL/Read CM Dict  Commented=on  xname=Traffic.T27.rzv  xsync=off  xstime=Inherited
  Read CM Dict17 : CarMaker4SL/Read CM Dict  Commented=on  xname=Traffic.T28.rzv  xsync=off  xstime=Inherited
  Read CM Dict18 : CarMaker4SL/Read CM Dict  Commented=on  xname=Car.Fr1.tx  xsync=off  xstime=Inherited
  Read CM Dict19 : CarMaker4SL/Read CM Dict  Commented=on  xname=Car.Fr1.ty  xsync=off  xstime=Inherited
  Read CM Dict2 : CarMaker4SL/Read CM Dict  Commented=on  xname=Traffic.T23.rzv  xsync=off  xstime=Inherited
  Read CM Dict20 : CarMaker4SL/Read CM Dict  Commented=on  xname=Car.v  xsync=off  xstime=Inherited
  Read CM Dict21 : CarMaker4SL/Read CM Dict  Commented=on  xname=Car.Fr1.rz  xsync=off  xstime=Inherited
  Read CM Dict22 : CarMaker4SL/Read CM Dict  Commented=on  xname=Traffic.T21.rzv  xsync=off  xstime=Inherited
  Read CM Dict23 : CarMaker4SL/Read CM Dict  Commented=on  xname=Traffic.T22.rzv  xsync=off  xstime=Inherited
  Read CM Dict24 : CarMaker4SL/Read CM Dict  Commented=on  xname=Traffic.T23.rzv  xsync=off  xstime=Inherited
  Read CM Dict25 : CarMaker4SL/Read CM Dict  Commented=on  xname=Traffic.T24.rzv  xsync=off  xstime=Inherited
  Read CM Dict26 : CarMaker4SL/Read CM Dict  Commented=on  xname=Traffic.T25.rzv  xsync=off  xstime=Inherited
  Read CM Dict27 : CarMaker4SL/Read CM Dict  Commented=on  xname=Traffic.T26.rzv  xsync=off  xstime=Inherited
  Read CM Dict28 : CarMaker4SL/Read CM Dict  Commented=on  xname=Traffic.T27.rzv  xsync=off  xstime=Inherited
  Read CM Dict29 : CarMaker4SL/Read CM Dict  Commented=on  xname=Traffic.T28.rzv  xsync=off  xstime=Inherited
  Read CM Dict3 : CarMaker4SL/Read CM Dict  Commented=on  xname=Traffic.T24.rzv  xsync=off  xstime=Inherited
  Read CM Dict30 : CarMaker4SL/Read CM Dict  Commented=on  xname=Car.ax  xsync=off  xstime=Inherited
  Read CM Dict31 : CarMaker4SL/Read CM Dict  xname=Car.Fr1.tx  xsync=off  xstime=Inherited
  Read CM Dict32 : CarMaker4SL/Read CM Dict  xname=Car.Fr1.ty  xsync=off  xstime=Inherited
  Read CM Dict4 : CarMaker4SL/Read CM Dict  Commented=on  xname=Car.Road.Path.DevDist  xsync=off  xstime=Inherited
  Read CM Dict5 : CarMaker4SL/Read CM Dict  Commented=on  xname=Car.Fr1.tx  xsync=off  xstime=Inherited
  Read CM Dict6 : CarMaker4SL/Read CM Dict  Commented=on  xname=Car.Fr1.ty  xsync=off  xstime=Inherited
  Read CM Dict7 : CarMaker4SL/Read CM Dict  Commented=on  xname=Car.v  xsync=off  xstime=Inherited
  Read CM Dict8 : CarMaker4SL/Read CM Dict  Commented=on  xname=Car.Fr1.rz  xsync=off  xstime=Inherited
  Read CM Dict9 : CarMaker4SL/Read CM Dict  Commented=on  xname=Car.ax  xsync=off  xstime=Inherited
  Reshape1 : Reshape  Commented=on  OutputDimensionality=Row vector (2-D)  OutputDimensions=[2,2]
  Saturation1 : Saturate  Commented=on  UpperLimit=0.7  LowerLimit=-0.7
  Saturation2 : Saturate  Commented=on  UpperLimit=1  LowerLimit=-1
  Saturation3 : Saturate  Commented=on  UpperLimit=0.7  LowerLimit=-0.7
  Scope{,1..2,5..6,8} (6 alike) : Scope  Commented=on
  Scope3 : Scope
  Scope4 : Scope
  Subsystem : Subsystem  Commented=on
  Terminator{,1..60} (61 alike) : Terminator  Commented=on
  To Workspace : ToWorkspace  Commented=on  VariableName=Trajectory_path  SaveFormat=Timeseries  SampleTime=-1
  To Workspace1 : ToWorkspace  Commented=on  VariableName=localll  SaveFormat=Timeseries  SampleTime=-1
  To Workspace2 : ToWorkspace  Commented=on  VariableName=Trajectory_path1  SaveFormat=Timeseries  SampleTime=-1
  To Workspace3 : ToWorkspace  Commented=on  VariableName=localll1  SaveFormat=Timeseries  SampleTime=-1
  Traffic Object : CarMaker4SL/Traffic Object  Commented=on  xname=T00  ximode=Traffic Id  xstime=Inherited
      settings: SourceProductName=CarMaker4SL
  Traffic Object1 : CarMaker4SL/Traffic Object  Commented=on  xname=T01  ximode=Traffic Id  xstime=Inherited
      settings: SourceProductName=CarMaker4SL
  Traffic Object10 : CarMaker4SL/Traffic Object  Commented=on  xname=T11  ximode=Traffic Id  xstime=Inherited
      settings: SourceProductName=CarMaker4SL
  Traffic Object11 : CarMaker4SL/Traffic Object  Commented=on  xname=T12  ximode=Traffic Id  xstime=Inherited
      settings: SourceProductName=CarMaker4SL
  Traffic Object12 : CarMaker4SL/Traffic Object  Commented=on  xname=T13  ximode=Traffic Id  xstime=Inherited
      settings: SourceProductName=CarMaker4SL
  Traffic Object13 : CarMaker4SL/Traffic Object  Commented=on  xname=T14  ximode=Traffic Id  xstime=Inherited
      settings: SourceProductName=CarMaker4SL
  Traffic Object14 : CarMaker4SL/Traffic Object  Commented=on  xname=T15  ximode=Traffic Id  xstime=Inherited
      settings: SourceProductName=CarMaker4SL
  Traffic Object15 : CarMaker4SL/Traffic Object  Commented=on  xname=T16  ximode=Traffic Id  xstime=Inherited
      settings: SourceProductName=CarMaker4SL
  Traffic Object16 : CarMaker4SL/Traffic Object  Commented=on  xname=T17  ximode=Traffic Id  xstime=Inherited
      settings: SourceProductName=CarMaker4SL
  Traffic Object17 : CarMaker4SL/Traffic Object  Commented=on  xname=T18  ximode=Traffic Id  xstime=Inherited
      settings: SourceProductName=CarMaker4SL
  Traffic Object18 : CarMaker4SL/Traffic Object  Commented=on  xname=T19  ximode=Traffic Id  xstime=Inherited
      settings: SourceProductName=CarMaker4SL
  Traffic Object19 : CarMaker4SL/Traffic Object  Commented=on  xname=T06  ximode=Traffic Id  xstime=Inherited
      settings: SourceProductName=CarMaker4SL
  Traffic Object2 : CarMaker4SL/Traffic Object  Commented=on  xname=T02  ximode=Traffic Id  xstime=Inherited
      settings: SourceProductName=CarMaker4SL
  Traffic Object20 : CarMaker4SL/Traffic Object  Commented=on  xname=T20  ximode=Traffic Id  xstime=Inherited
      settings: SourceProductName=CarMaker4SL
  Traffic Object21 : CarMaker4SL/Traffic Object  Commented=on  xname=T21  ximode=Traffic Id  xstime=Inherited
      settings: SourceProductName=CarMaker4SL
  Traffic Object22 : CarMaker4SL/Traffic Object  Commented=on  xname=T22  ximode=Traffic Id  xstime=Inherited
      settings: SourceProductName=CarMaker4SL
  Traffic Object23 : CarMaker4SL/Traffic Object  Commented=on  xname=T23  ximode=Traffic Id  xstime=Inherited
      settings: SourceProductName=CarMaker4SL
  Traffic Object24 : CarMaker4SL/Traffic Object  Commented=on  xname=T24  ximode=Traffic Id  xstime=Inherited
      settings: SourceProductName=CarMaker4SL
  Traffic Object25 : CarMaker4SL/Traffic Object  Commented=on  xname=T25  ximode=Traffic Id  xstime=Inherited
      settings: SourceProductName=CarMaker4SL
  Traffic Object26 : CarMaker4SL/Traffic Object  Commented=on  xname=T26  ximode=Traffic Id  xstime=Inherited
      settings: SourceProductName=CarMaker4SL
  Traffic Object27 : CarMaker4SL/Traffic Object  Commented=on  xname=T27  ximode=Traffic Id  xstime=Inherited
      settings: SourceProductName=CarMaker4SL
  Traffic Object28 : CarMaker4SL/Traffic Object  Commented=on  xname=T28  ximode=Traffic Id  xstime=Inherited
      settings: SourceProductName=CarMaker4SL
  Traffic Object29 : CarMaker4SL/Traffic Object  Commented=on  xname=T08  ximode=Traffic Id  xstime=Inherited
      settings: SourceProductName=CarMaker4SL
  Traffic Object3 : CarMaker4SL/Traffic Object  Commented=on  xname=T00  ximode=Traffic Id  xstime=Inherited
      settings: SourceProductName=CarMaker4SL
  Traffic Object30 : CarMaker4SL/Traffic Object  Commented=on  xname=T09  ximode=Traffic Id  xstime=Inherited
      settings: SourceProductName=CarMaker4SL
  Traffic Object31 : CarMaker4SL/Traffic Object  Commented=on  xname=T10  ximode=Traffic Id  xstime=Inherited
      settings: SourceProductName=CarMaker4SL
  Traffic Object32 : CarMaker4SL/Traffic Object  Commented=on  xname=T11  ximode=Traffic Id  xstime=Inherited
      settings: SourceProductName=CarMaker4SL
  Traffic Object33 : CarMaker4SL/Traffic Object  Commented=on  xname=T12  ximode=Traffic Id  xstime=Inherited
      settings: SourceProductName=CarMaker4SL
  Traffic Object34 : CarMaker4SL/Traffic Object  Commented=on  xname=T13  ximode=Traffic Id  xstime=Inherited
      settings: SourceProductName=CarMaker4SL
  Traffic Object35 : CarMaker4SL/Traffic Object  Commented=on  xname=T14  ximode=Traffic Id  xstime=Inherited
      settings: SourceProductName=CarMaker4SL
  Traffic Object36 : CarMaker4SL/Traffic Object  Commented=on  xname=T15  ximode=Traffic Id  xstime=Inherited
      settings: SourceProductName=CarMaker4SL
  Traffic Object37 : CarMaker4SL/Traffic Object  Commented=on  xname=T16  ximode=Traffic Id  xstime=Inherited
      settings: SourceProductName=CarMaker4SL
  Traffic Object38 : CarMaker4SL/Traffic Object  Commented=on  xname=T17  ximode=Traffic Id  xstime=Inherited
      settings: SourceProductName=CarMaker4SL
  Traffic Object39 : CarMaker4SL/Traffic Object  Commented=on  xname=T18  ximode=Traffic Id  xstime=Inherited
      settings: SourceProductName=CarMaker4SL
  Traffic Object4 : CarMaker4SL/Traffic Object  Commented=on  xname=T01  ximode=Traffic Id  xstime=Inherited
      settings: SourceProductName=CarMaker4SL
  Traffic Object40 : CarMaker4SL/Traffic Object  Commented=on  xname=T19  ximode=Traffic Id  xstime=Inherited
      settings: SourceProductName=CarMaker4SL
  Traffic Object41 : CarMaker4SL/Traffic Object  Commented=on  xname=T06  ximode=Traffic Id  xstime=Inherited
      settings: SourceProductName=CarMaker4SL
  Traffic Object42 : CarMaker4SL/Traffic Object  Commented=on  xname=T20  ximode=Traffic Id  xstime=Inherited
      settings: SourceProductName=CarMaker4SL
  Traffic Object43 : CarMaker4SL/Traffic Object  Commented=on  xname=T21  ximode=Traffic Id  xstime=Inherited
      settings: SourceProductName=CarMaker4SL
  Traffic Object44 : CarMaker4SL/Traffic Object  Commented=on  xname=T22  ximode=Traffic Id  xstime=Inherited
      settings: SourceProductName=CarMaker4SL
  Traffic Object45 : CarMaker4SL/Traffic Object  Commented=on  xname=T23  ximode=Traffic Id  xstime=Inherited
      settings: SourceProductName=CarMaker4SL
  Traffic Object46 : CarMaker4SL/Traffic Object  Commented=on  xname=T24  ximode=Traffic Id  xstime=Inherited
      settings: SourceProductName=CarMaker4SL
  Traffic Object47 : CarMaker4SL/Traffic Object  Commented=on  xname=T25  ximode=Traffic Id  xstime=Inherited
      settings: SourceProductName=CarMaker4SL
  Traffic Object48 : CarMaker4SL/Traffic Object  Commented=on  xname=T26  ximode=Traffic Id  xstime=Inherited
      settings: SourceProductName=CarMaker4SL
  Traffic Object49 : CarMaker4SL/Traffic Object  Commented=on  xname=T27  ximode=Traffic Id  xstime=Inherited
      settings: SourceProductName=CarMaker4SL
  Traffic Object5 : CarMaker4SL/Traffic Object  Commented=on  xname=T02  ximode=Traffic Id  xstime=Inherited
      settings: SourceProductName=CarMaker4SL
  Traffic Object50 : CarMaker4SL/Traffic Object  Commented=on  xname=T28  ximode=Traffic Id  xstime=Inherited
      settings: SourceProductName=CarMaker4SL
  Traffic Object51 : CarMaker4SL/Traffic Object  Commented=on  xname=T08  ximode=Traffic Id  xstime=Inherited
      settings: SourceProductName=CarMaker4SL
  Traffic Object52 : CarMaker4SL/Traffic Object  Commented=on  xname=T00  ximode=Traffic Id  xstime=Inherited
      settings: SourceProductName=CarMaker4SL
  Traffic Object53 : CarMaker4SL/Traffic Object  Commented=on  xname=T09  ximode=Traffic Id  xstime=Inherited
      settings: SourceProductName=CarMaker4SL
  Traffic Object54 : CarMaker4SL/Traffic Object  Commented=on  xname=T10  ximode=Traffic Id  xstime=Inherited
      settings: SourceProductName=CarMaker4SL
  Traffic Object55 : CarMaker4SL/Traffic Object  Commented=on  xname=T01  ximode=Traffic Id  xstime=Inherited
      settings: SourceProductName=CarMaker4SL
  Traffic Object56 : CarMaker4SL/Traffic Object  Commented=on  xname=T02  ximode=Traffic Id  xstime=Inherited
      settings: SourceProductName=CarMaker4SL
  Traffic Object57 : CarMaker4SL/Traffic Object  Commented=on  xname=T03  ximode=Traffic Id  xstime=Inherited
      settings: SourceProductName=CarMaker4SL
  Traffic Object58 : CarMaker4SL/Traffic Object  Commented=on  xname=T04  ximode=Traffic Id  xstime=Inherited
      settings: SourceProductName=CarMaker4SL
  Traffic Object59 : CarMaker4SL/Traffic Object  Commented=on  xname=T05  ximode=Traffic Id  xstime=Inherited
      settings: SourceProductName=CarMaker4SL
  Traffic Object6 : CarMaker4SL/Traffic Object  Commented=on  xname=T03  ximode=Traffic Id  xstime=Inherited
      settings: SourceProductName=CarMaker4SL
  Traffic Object60 : CarMaker4SL/Traffic Object  Commented=on  xname=T07  ximode=Traffic Id  xstime=Inherited
      settings: SourceProductName=CarMaker4SL
  Traffic Object7 : CarMaker4SL/Traffic Object  Commented=on  xname=T04  ximode=Traffic Id  xstime=Inherited
      settings: SourceProductName=CarMaker4SL
  Traffic Object8 : CarMaker4SL/Traffic Object  Commented=on  xname=T05  ximode=Traffic Id  xstime=Inherited
      settings: SourceProductName=CarMaker4SL
  Traffic Object9 : CarMaker4SL/Traffic Object  Commented=on  xname=T07  ximode=Traffic Id  xstime=Inherited
      settings: SourceProductName=CarMaker4SL
  Transpose{,1..25} (26 alike) : Math  Commented=on  Operator=transpose
  Unit Delay : UnitDelay  SampleTime=-1  HasFrameUpgradeWarning=on
  Unit Delay1 : UnitDelay  SampleTime=-1  HasFrameUpgradeWarning=on
  Unit Delay2 : UnitDelay  SampleTime=-1  HasFrameUpgradeWarning=on
  Write CM Dict1 : CarMaker4SL/Write CM Dict  Commented=on  xname=Car.CFL.rz_ext  xsync=off
  Write CM Dict2 : CarMaker4SL/Write CM Dict  Commented=on  xname=Car.CFR.rz_ext  xsync=off
  Write CM Dict3 : CarMaker4SL/Write CM Dict  Commented=on  xname=Car.CFL.rz_ext  xsync=off
  Write CM Dict4 : CarMaker4SL/Write CM Dict  Commented=on  xname=Car.CFR.rz_ext  xsync=off
  Write CM Dict5 : CarMaker4SL/Write CM Dict  Commented=on  xname=AccelCtrl.DesiredAx  xsync=off
  Write CM Dict6 : CarMaker4SL/Write CM Dict  Commented=on  xname=AccelCtrl.DesiredAx  xsync=off
  Write CM Dict7 : CarMaker4SL/Write CM Dict  Commented=on  xname=Car.CFL.rz_ext  xsync=off
  Write CM Dict8 : CarMaker4SL/Write CM Dict  Commented=on  xname=Car.CFR.rz_ext  xsync=off
  Write CM Dict9 : CarMaker4SL/Write CM Dict  Commented=on  xname=AccelCtrl.DesiredAx  xsync=off
  target lane_ Gate : Constant  Commented=on  Value=3
  target lane_ Gate1 : Constant  Commented=on  Value=3
  Traffic_Info : Outport
  Traffic_Info1 : Outport  Port=2
  wires:
  Constant1/1 -> Traffic Object/1
  Read CM Dict/1 -> Goto1/1
  Constant/1 -> Goto4/1
  Bus Selector/4 -> Goto7/1  "<v_0 y>"
  Traffic Object/1 -> Terminator/1
  Bus Selector/3 -> Goto6/1  "<v_0 x>"
  Traffic Object/2 -> Bus Selector/1
  Bus Selector/1 -> Goto3/1  "<t_0 x>"
  Bus Selector/2 -> Goto5/1  "<t_0 y>"
  Read CM Dict1/1 -> Goto2/1
  Bus Selector/5 -> Goto8/1  "<a_0 x>"
  Bus Selector/6 -> Goto9/1  "<a_0 y>"
  Bus Selector/7 -> Goto10/1  "<r_zyx z>"
  Read CM Dict2/1 -> Goto12/1
  Bus Selector1/1 -> Goto13/1  "<t_0 x>"
  Bus Selector1/5 -> Goto17/1  "<a_0 x>"
  Bus Selector1/6 -> Goto18/1  "<a_0 y>"
  Bus Selector1/7 -> Goto11/1  "<r_zyx z>"
  Traffic Object1/1 -> Terminator1/1
  Bus Selector1/4 -> Goto16/1  "<v_0 y>"
  Constant2/1 -> Traffic Object1/1
  Traffic Object1/2 -> Bus Selector1/1
  Bus Selector1/3 -> Goto15/1  "<v_0 x>"
  Bus Selector1/2 -> Goto14/1  "<t_0 y>"
  Bus Selector2/3 -> Goto23/1  "<v_0 x>"
  Bus Selector2/2 -> Goto22/1  "<t_0 y>"
  Traffic Object2/2 -> Bus Selector2/1
  Bus Selector2/1 -> Goto21/1  "<t_0 x>"
  Bus Selector2/6 -> Goto26/1  "<a_0 y>"
  Constant3/1 -> Traffic Object2/1
  Traffic Object2/1 -> Terminator2/1
  Bus Selector2/7 -> Goto19/1  "<r_zyx z>"
  Bus Selector2/5 -> Goto25/1  "<a_0 x>"
  Read CM Dict3/1 -> Goto20/1
  Bus Selector2/4 -> Goto24/1  "<v_0 y>"
  Constant10/1 -> Mux3/1
  Constant5/1 -> Mux3/2
  Reshape1/1 -> Goto28/1
  Mux3/1 -> Reshape1/1
  Subsystem/1(Traffic_Info) -> Goto30/1
  Read CM Dict4/1 -> Goto27/1
  Constant4/1 -> Goto29/1
  From5/1 -> Mux/2
  From54/1 -> Add/2
  Add/1 -> PID Controller1/1
  From3/1 -> "MATLAB Function4 "/3(head)
  PID Controller1/1 -> Write CM Dict5/1
  From7/1 -> MATLAB Function3/1(poly_coeff)
  Gain/1 -> Saturation1/1
  From57/1 -> To Workspace/1, "MATLAB Function4 "/1(waypoints)
  MATLAB Function4/1(poly_coeff) -> Goto36/1, Scope2/1
  Constant7/1 -> MATLAB Function3/3(lookahead_time)
  From6/1 -> MATLAB Function4/1(local_waypoints)
  From4/1 -> Mux/1
  From8/1 -> MATLAB Function3/2(velocity)
  Mux/1 -> "MATLAB Function4 "/2(vehicle_position)
  MATLAB Function3/1(lateral_error) -> Goto37/1
  Saturation1/1 -> Write CM Dict4/1, Write CM Dict3/1
  "MATLAB Function4 "/1(local_waypoints_) -> To Workspace1/1, Goto31/1
  PID Controller/1 -> Gain/1
  Constant6/1 -> Goto38/1
  Read CM Dict6/1 -> Goto33/1
  Constant8/1 -> Goto39/1
  Read CM Dict5/1 -> Goto32/1
  Read CM Dict7/1 -> Goto34/1
  Constant9/1 -> Goto40/1
  Read CM Dict8/1 -> Goto35/1
  MATLAB Function9/1(ego_lane_idx) -> Scope/1, Goto43/1
  From35/1 -> MATLAB Function9/4(wp2)
  From37/1 -> Mux2/1
  MATLAB Function9/2(traffic_lane_idx) -> Scope6/1, Goto42/1
  From36/1 -> MATLAB Function9/5(wp3)
  From34/1 -> MATLAB Function9/3(wp1)
  From38/1 -> Mux2/2
  Mux6/1 -> MATLAB Function11/1(ego_pos)
  Rate Limiter/1 -> Goto45/1
  MATLAB Function11/2(debug_time_gap) -> Scope8/1
  MATLAB Function11/1(target_speed) -> Rate Limiter/1
  From71/1 -> MATLAB Function11/3(ego_vx)
  From65/1 -> MATLAB Function11/2(ego_yaw)
  From67/1 -> MATLAB Function11/6(traffic_lane_idx)
  From66/1 -> MATLAB Function11/4(ego_lane_idx)
  From63/1 -> Mux6/1
  From64/1 -> Mux6/2
  From48/1 -> Transpose/1
  From49/1 -> Transpose1/1
  From50/1 -> Transpose2/1
  From51/1 -> Transpose3/1
  From52/1 -> Transpose4/1
  From53/1 -> Transpose5/1
  From56/1 -> Transpose6/1
  From72/1 -> Transpose7/1
  Matrix Concatenate/1 -> MATLAB Function11/5(traffic_info), MATLAB Function9/2(traffic_info)
  Constant105/1 -> Mux63/2
  Mux67/1 -> Mux66/2
  Constant103/1 -> Mux69/2
  Constant98/1 -> Mux63/1
  Constant102/1 -> Mux69/1
  Mux63/1 -> Mux66/1
  Constant100/1 -> Mux68/1
  Mux68/1 -> Mux66/3
  Constant99/1 -> Mux67/2
  Constant104/1 -> Mux67/1
  Mux69/1 -> Mux66/4
  Constant101/1 -> Mux68/2
  Mux66/1 -> Goto74/1
  Mux47/1 -> Mux46/4
  Constant91/1 -> Traffic Object3/1
  Bus Selector31/6 -> Mux64/6  "<a_0 y>"
  Mux44/1 -> Goto59/1
  Traffic Object20/1 -> Terminator20/1
  Constant81/1 -> Traffic Object26/1
  From17/1 -> Mux59/18
  Bus Selector13/3 -> Mux26/3  "<r_zyx z>"
  From39/1 -> Mux59/28
  From21/1 -> Mux59/21
  From45/1 -> Mux59/8
  Bus Selector4/1 -> Mux5/1  "<t_0 x>"
  Bus Selector30/2 -> Mux18/2  "<t_0 y>"
  Bus Selector11/1 -> Mux20/1  "<t_0 x>"
  Constant51/1 -> Traffic Object17/1
  Bus Selector30/3 -> Mux18/3  "<r_zyx z>"
  Traffic Object7/1 -> Terminator7/1
  Traffic Object16/1 -> Terminator16/1
  Bus Selector18/3 -> Mux38/3  "<r_zyx z>"
  Traffic Object19/2 -> Bus Selector19/1
  From20/1 -> Mux59/3
  From22/1 -> Mux59/22
  Bus Selector3/3 -> Mux1/3  "<r_zyx z>"
  Mux46/1 -> Goto58/1
  Bus Selector12/3 -> Mux24/3  "<r_zyx z>"
  Traffic Object17/1 -> Terminator17/1
  From15/1 -> Mux59/16
  Bus Selector31/5 -> Mux64/5  "<a_0 x>"
  Mux31/1 -> Mux30/4
  Traffic Object27/2 -> Bus Selector27/1
  Mux21/1 -> Mux20/4
  Constant17/1 -> Mux11/2
  Bus Selector10/1 -> Mux22/1  "<t_0 x>"
  Traffic Object17/2 -> Bus Selector16/1
  Bus Selector17/2 -> Mux34/2  "<t_0 y>"
  Constant56/1 -> Mux35/1
  Constant41/1 -> Traffic Object14/1
  Bus Selector17/3 -> Mux34/3  "<r_zyx z>"
  Bus Selector26/1 -> Mux54/1  "<t_0 x>"
  Constant20/1 -> Traffic Object7/1
  Mux34/1 -> Goto52/1
  Read CM Dict26/1 -> Mux48/8
  Bus Selector21/1 -> Mux42/1  "<t_0 x>"
  Mux50/1 -> Goto61/1
  Mux16/1 -> Goto71/1
  Traffic Object10/1 -> Terminator10/1
  Mux5/1 -> Goto55/1
  Bus Selector11/2 -> Mux20/2  "<t_0 y>"
  Mux42/1 -> Goto57/1
  From40/1 -> Mux59/29
  Bus Selector13/1 -> Mux26/1  "<t_0 x>"
  Bus Selector27/3 -> Mux52/3  "<v_0 x>"
  Constant42/1 -> Mux27/1
  Mux30/1 -> Goto49/1
  Constant66/1 -> Mux8/2
  Traffic Object23/2 -> Bus Selector23/1
  Mux29/1 -> Mux28/4
  Mux27/1 -> Mux26/4
  Constant49/1 -> Mux29/2
  Bus Selector21/2 -> Mux42/2  "<t_0 y>"
  Bus Selector27/6 -> Mux52/6  "<a_0 y>"
  Bus Selector12/1 -> Mux24/1  "<t_0 x>"
  Bus Selector6/1 -> Mux57/1  "<t_0 x>"
  Traffic Object11/1 -> Terminator11/1
  Bus Selector12/2 -> Mux24/2  "<t_0 y>"
  Traffic Object16/2 -> Bus Selector18/1
  Traffic Object21/2 -> Bus Selector20/1
  Traffic Object29/2 -> Bus Selector9/1
  Constant63/1 -> Mux39/2
  Traffic Object14/1 -> Terminator14/1
  Bus Selector9/3 -> Mux12/3  "<r_zyx z>"
  Constant19/1 -> Mux13/1
  Bus Selector18/1 -> Mux38/1  "<t_0 x>"
  Bus Selector16/2 -> Mux32/2  "<t_0 y>"
  From47/1 -> Mux59/10
  Constant34/1 -> Traffic Object30/1
  Constant88/1 -> Mux56/1
  Bus Selector28/3 -> Mux16/3  "<r_zyx z>"
  Bus Selector19/1 -> Mux36/1  "<t_0 x>"
  Bus Selector7/2 -> Mux10/2  "<t_0 y>"
  Mux19/1 -> Mux18/4
  Constant52/1 -> Mux33/1
  Traffic Object29/1 -> Terminator29/1
  Traffic Object10/2 -> Bus Selector30/1
  Mux39/1 -> Mux38/4
  Bus Selector4/3 -> Mux5/3  "<r_zyx z>"
  Bus Selector8/1 -> Mux14/1  "<t_0 x>"
  Bus Selector16/1 -> Mux32/1  "<t_0 x>"
  Constant95/1 -> Traffic Object28/1
  Traffic Object8/1 -> Terminator8/1
  Constant61/1 -> Mux39/1
  Mux38/1 -> Goto53/1
  Constant38/1 -> Traffic Object13/1
  Bus Selector29/1 -> Mux60/1  "<t_0 x>"
  From41/1 -> Mux59/4
  Constant46/1 -> Mux29/1
  From13/1 -> Mux59/14
  Mux33/1 -> Mux32/4
  Bus Selector27/1 -> Mux52/1  "<t_0 x>"
  Traffic Object5/2 -> Bus Selector4/1
  Mux17/1 -> Mux16/4
  Bus Selector23/6 -> Mux44/6  "<a_0 y>"
  From/1 -> Mux59/1
  Traffic Object3/1 -> Terminator3/1
  Bus Selector11/3 -> Mux20/3  "<r_zyx z>"
  Traffic Object31/2 -> Bus Selector28/1
  Constant40/1 -> Mux25/2
  Mux48/1 -> Goto60/1
  Bus Selector14/3 -> Mux30/3  "<r_zyx z>"
  Traffic Object7/2 -> Bus Selector8/1
  Bus Selector24/4 -> Mux48/4  "<v_0 y>"
  Constant26/1 -> Mux17/1
  Mux20/1 -> Goto46/1
  Constant36/1 -> Mux21/2
  Bus Selector20/2 -> Mux40/2  "<t_0 y>"
  Bus Selector9/2 -> Mux12/2  "<t_0 y>"
  Constant31/1 -> Traffic Object11/1
  Bus Selector10/2 -> Mux22/2  "<t_0 y>"
  Constant32/1 -> Mux21/1
  Bus Selector28/1 -> Mux16/1  "<t_0 x>"
  Mux65/1 -> Mux64/9
  Bus Selector26/2 -> Mux54/2  "<t_0 y>"
  Constant15/1 -> Traffic Object9/1
  Bus Selector9/1 -> Mux12/1  "<t_0 x>"
  Constant54/1 -> Traffic Object18/1
  Traffic Object30/2 -> Bus Selector10/1
  Traffic Object9/2 -> Bus Selector7/1
  Traffic Object15/2 -> Bus Selector15/1
  Constant22/1 -> Mux4/1
  Constant16/1 -> Mux11/1
  Mux4/1 -> Mux1/4
  Bus Selector15/3 -> Mux28/3  "<r_zyx z>"
  Traffic Object8/2 -> Bus Selector6/1
  Traffic Object18/2 -> Bus Selector17/1
  Bus Selector6/3 -> Mux57/3  "<r_zyx z>"
  Mux23/1 -> Mux22/4
  Constant37/1 -> Mux23/2
  Traffic Object30/1 -> Terminator30/1
  Bus Selector8/2 -> Mux14/2  "<t_0 y>"
  Traffic Object9/1 -> Terminator9/1
  Constant77/1 -> Traffic Object6/1
  Bus Selector25/3 -> Mux50/3  "<v_0 x>"
  Mux13/1 -> Mux12/4
  Bus Selector18/2 -> Mux38/2  "<t_0 y>"
  Constant23/1 -> Mux13/2
  Constant21/1 -> Mux15/1
  Bus Selector20/3 -> Mux40/3  "<v_0 x>"
  Constant65/1 -> Mux41/1
  Constant13/1 -> Mux58/1
  Bus Selector6/2 -> Mux57/2  "<t_0 y>"
  Constant28/1 -> Traffic Object10/1
  Mux15/1 -> Mux14/4
  Bus Selector30/1 -> Mux18/1  "<t_0 x>"
  Constant60/1 -> Traffic Object16/1
  Constant18/1 -> Traffic Object29/1
  Bus Selector24/5 -> Mux48/5  "<a_0 x>"
  Mux9/1 -> Goto65/1
  Constant48/1 -> Mux31/1
  Bus Selector5/2 -> Mux9/2  "<t_0 y>"
  Mux61/1 -> Mux60/4
  Constant53/1 -> Mux33/2
  Constant85/1 -> Mux53/1
  Constant12/1 -> Traffic Object8/1
  Bus Selector8/3 -> Mux14/3  "<r_zyx z>"
  From43/1 -> Mux59/6
  Bus Selector31/3 -> Mux64/3  "<v_0 x>"
  Constant14/1 -> Mux58/2
  Mux56/1 -> Mux9/4
  Bus Selector5/1 -> Mux9/1  "<t_0 x>"
  From26/1 -> Mux59/26
  Mux58/1 -> Mux57/4
  Bus Selector15/1 -> Mux28/1  "<t_0 x>"
  Traffic Object6/2 -> Bus Selector5/1
  Mux64/1 -> Goto66/1
  From1/1 -> Mux59/2
  Constant44/1 -> Traffic Object5/1
  Bus Selector23/5 -> Mux44/5  "<a_0 x>"
  Mux8/1 -> Mux5/4
  From25/1 -> Mux59/25
  Read CM Dict29/1 -> Mux64/8
  Traffic Object5/1 -> Terminator5/1
  Traffic Object28/2 -> Bus Selector31/1
  Bus Selector31/2 -> Mux64/2  "<t_0 y>"
  Constant47/1 -> Traffic Object12/1
  Bus Selector3/2 -> Mux1/2  "<t_0 y>"
  Constant11/1 -> Traffic Object4/1
  From12/1 -> Mux59/13
  Mux14/1 -> Goto69/1
  Traffic Object12/2 -> Bus Selector14/1
  Traffic Object4/1 -> Terminator4/1
  Constant74/1 -> Mux47/1
  Traffic Object28/1 -> Terminator28/1
  Constant87/1 -> Mux55/1
  Bus Selector31/1 -> Mux64/1  "<t_0 x>"
  Bus Selector13/2 -> Mux26/2  "<t_0 y>"
  Constant90/1 -> Mux55/2
  Constant89/1 -> Mux53/2
  Constant45/1 -> Traffic Object15/1
  Bus Selector31/7 -> Mux64/7  "<r_zyx z>"
  Constant80/1 -> Mux49/2
  Bus Selector22/2 -> Mux46/2  "<t_0 y>"
  Mux41/1 -> Mux40/9
  Traffic Object25/1 -> Terminator25/1
  Constant82/1 -> Mux51/1
  Bus Selector25/7 -> Mux50/7  "<r_zyx z>"
  Bus Selector7/3 -> Mux10/3  "<r_zyx z>"
  Bus Selector24/2 -> Mux48/2  "<t_0 y>"
  From42/1 -> Mux59/5
  Mux24/1 -> Goto47/1
  Constant57/1 -> Mux35/2
  Read CM Dict25/1 -> Mux54/8
  Constant67/1 -> Mux41/2
  Bus Selector27/7 -> Mux52/7  "<r_zyx z>"
  Constant78/1 -> Traffic Object25/1
  From19/1 -> Mux59/20
  Constant96/1 -> Mux65/1
  From44/1 -> Mux59/7
  Bus Selector24/6 -> Mux48/6  "<a_0 y>"
  Bus Selector27/4 -> Mux52/4  "<v_0 y>"
  Constant24/1 -> Mux15/2
  Mux28/1 -> Goto50/1
  Constant86/1 -> Traffic Object24/1
  Bus Selector26/4 -> Mux54/4  "<v_0 y>"
  Bus Selector25/1 -> Mux50/1  "<t_0 x>"
  Mux52/1 -> Goto63/1
  Mux53/1 -> Mux52/9
  Read CM Dict28/1 -> Mux52/8
  Traffic Object4/2 -> Bus Selector3/1
  Traffic Object12/1 -> Terminator12/1
  Traffic Object24/1 -> Terminator24/1
  Bus Selector23/3 -> Mux44/3  "<v_0 x>"
  From24/1 -> Mux59/24
  Bus Selector26/7 -> Mux54/7  "<r_zyx z>"
  Read CM Dict24/1 -> Mux44/8
  Traffic Object26/1 -> Terminator26/1
  Bus Selector22/3 -> Mux46/3  "<r_zyx z>"
  Bus Selector27/5 -> Mux52/5  "<a_0 x>"
  Traffic Object15/1 -> Terminator15/1
  Bus Selector25/2 -> Mux50/2  "<t_0 y>"
  Traffic Object11/2 -> Bus Selector11/1
  Bus Selector21/3 -> Mux42/3  "<v_0 x>"
  Bus Selector27/2 -> Mux52/2  "<t_0 y>"
  Bus Selector3/1 -> Mux1/1  "<t_0 x>"
  Bus Selector25/5 -> Mux50/5  "<a_0 x>"
  Mux54/1 -> Goto62/1
  Bus Selector20/4 -> Mux40/4  "<v_0 y>"
  From18/1 -> Mux59/19
  From11/1 -> Mux59/12
  Bus Selector26/6 -> Mux54/6  "<a_0 y>"
  Bus Selector7/1 -> Mux10/1  "<t_0 x>"
  Bus Selector20/7 -> Mux40/7  "<r_zyx z>"
  Bus Selector24/1 -> Mux48/1  "<t_0 x>"
  Read CM Dict23/1 -> Mux42/8
  Traffic Object21/1 -> Terminator21/1
  Constant29/1 -> Mux19/1
  Constant43/1 -> Mux27/2
  Bus Selector20/5 -> Mux40/5  "<a_0 x>"
  Constant71/1 -> Traffic Object23/1
  Traffic Object22/1 -> Terminator22/1
  Bus Selector29/2 -> Mux60/2  "<t_0 y>"
  Constant72/1 -> Mux45/1
  Constant25/1 -> Traffic Object31/1
  Bus Selector20/1 -> Mux40/1  "<t_0 x>"
  Traffic Object27/1 -> Terminator27/1
  Bus Selector21/7 -> Mux42/7  "<r_zyx z>"
  Mux51/1 -> Mux50/9
  Constant50/1 -> Mux31/2
  Traffic Object6/1 -> Terminator6/1
  Constant64/1 -> Traffic Object21/1
  From46/1 -> Mux59/9
  Mux59/1 -> Traffic_Info/1
  Mux57/1 -> Goto67/1
  Bus Selector10/3 -> Mux22/3  "<r_zyx z>"
  Mux36/1 -> Goto54/1
  Constant69/1 -> Mux43/1
  Bus Selector23/4 -> Mux44/4  "<v_0 y>"
  Mux55/1 -> Mux54/9
  Constant94/1 -> Mux61/2
  Bus Selector20/6 -> Mux40/6  "<a_0 y>"
  From16/1 -> Mux59/17
  Bus Selector21/6 -> Mux42/6  "<a_0 y>"
  Mux11/1 -> Mux10/4
  Constant93/1 -> Mux56/2
  Mux35/1 -> Mux34/4
  Traffic Object20/2 -> Bus Selector22/1
  Mux40/1 -> Goto56/1
  Constant83/1 -> Mux51/2
  Bus Selector21/5 -> Mux42/5  "<a_0 x>"
  Traffic Object14/2 -> Bus Selector13/1
  Constant75/1 -> Mux45/2
  Bus Selector28/2 -> Mux16/2  "<t_0 y>"
  Traffic Object23/1 -> Terminator23/1
  Constant70/1 -> Mux43/2
  Mux10/1 -> Goto68/1
  Read CM Dict22/1 -> Mux40/8
  Traffic Object22/2 -> Bus Selector21/1
  Traffic Object25/2 -> Bus Selector24/1
  Constant92/1 -> Mux61/1
  Mux60/1 -> Goto64/1
  Bus Selector29/3 -> Mux60/3  "<r_zyx z>"
  Bus Selector24/3 -> Mux48/3  "<v_0 x>"
  Traffic Object13/2 -> Bus Selector12/1
  Constant30/1 -> Mux19/2
  Mux26/1 -> Goto48/1
  Mux43/1 -> Mux42/9
  Mux22/1 -> Goto44/1
  Constant76/1 -> Mux47/2
  Bus Selector4/2 -> Mux5/2  "<t_0 y>"
  From10/1 -> Mux59/11
  Bus Selector19/2 -> Mux36/2  "<t_0 y>"
  Bus Selector15/2 -> Mux28/2  "<t_0 y>"
  Constant27/1 -> Mux17/2
  Traffic Object3/2 -> Bus Selector29/1
  Traffic Object19/1 -> Terminator19/1
  Constant58/1 -> Traffic Object19/1
  Traffic Object24/2 -> Bus Selector26/1
  Traffic Object26/2 -> Bus Selector25/1
  Traffic Object13/1 -> Terminator13/1
  Mux45/1 -> Mux44/9
  Bus Selector31/4 -> Mux64/4  "<v_0 y>"
  Bus Selector23/7 -> Mux44/7  "<r_zyx z>"
  Traffic Object18/1 -> Terminator18/1
  Mux37/1 -> Mux36/4
  Bus Selector26/5 -> Mux54/5  "<a_0 x>"
  Bus Selector23/2 -> Mux44/2  "<t_0 y>"
  Constant73/1 -> Traffic Object20/1
  Mux12/1 -> Goto70/1
  Constant84/1 -> Traffic Object27/1
  Mux32/1 -> Goto51/1
  Bus Selector21/4 -> Mux42/4  "<v_0 y>"
  Bus Selector22/1 -> Mux46/1  "<t_0 x>"
  Bus Selector25/4 -> Mux50/4  "<v_0 y>"
  Constant55/1 -> Mux8/1
  Constant39/1 -> Mux25/1
  Bus Selector23/1 -> Mux44/1  "<t_0 x>"
  From14/1 -> Mux59/15
  Constant62/1 -> Mux37/2
  Constant59/1 -> Mux37/1
  Mux25/1 -> Mux24/4
  Bus Selector25/6 -> Mux50/6  "<a_0 y>"
  Read CM Dict27/1 -> Mux50/8
  Mux49/1 -> Mux48/9
  Bus Selector14/1 -> Mux30/1  "<t_0 x>"
  Bus Selector19/3 -> Mux36/3  "<r_zyx z>"
  Bus Selector5/3 -> Mux9/3  "<r_zyx z>"
  Constant68/1 -> Traffic Object22/1
  Constant33/1 -> Mux4/2
  Bus Selector16/3 -> Mux32/3  "<r_zyx z>"
  Bus Selector24/7 -> Mux48/7  "<r_zyx z>"
  Constant97/1 -> Mux65/2
  Bus Selector26/3 -> Mux54/3  "<v_0 x>"
  Mux18/1 -> Goto72/1
  Bus Selector17/1 -> Mux34/1  "<t_0 x>"
  Mux1/1 -> Goto41/1
  Bus Selector14/2 -> Mux30/2  "<t_0 y>"
  From23/1 -> Mux59/23
  Traffic Object31/1 -> Terminator31/1
  Constant79/1 -> Mux49/1
  Constant35/1 -> Mux23/1
  From27/1 -> Mux59/27
  Transpose/1 -> Matrix Concatenate/1
  Transpose1/1 -> Matrix Concatenate/2
  Transpose2/1 -> Matrix Concatenate/3
  Transpose3/1 -> Matrix Concatenate/4
  Transpose4/1 -> Matrix Concatenate/5
  Transpose6/1 -> Matrix Concatenate/7
  Transpose7/1 -> Matrix Concatenate/8
  Transpose5/1 -> Matrix Concatenate/6
  Constant106/1 -> Goto73/1
  From9/1 -> PID Controller/1
  From70/1 -> Transpose15/1
  Transpose13/1 -> Matrix Concatenate2/6
  Transpose15/1 -> Matrix Concatenate2/8
  Transpose14/1 -> Matrix Concatenate2/7
  Transpose11/1 -> Matrix Concatenate2/4
  Transpose12/1 -> Matrix Concatenate2/5
  Transpose9/1 -> Matrix Concatenate2/2
  Transpose10/1 -> Matrix Concatenate2/3
  From61/1 -> Transpose11/1
  From58/1 -> Transpose8/1
  Transpose8/1 -> Matrix Concatenate2/1
  From68/1 -> Transpose13/1
  From60/1 -> Transpose10/1
  From62/1 -> Transpose12/1
  From59/1 -> Transpose9/1
  From69/1 -> Transpose14/1
  Matrix Concatenate2/1 -> Goto/1
  From73/1 -> MATLAB Function7/1(global_waypoint)
  MATLAB Function7/1(s_ref) -> Goto76/1
  From74/1 -> MATLAB Function2/2(global_waypoint_2)
  From75/1 -> MATLAB Function2/1(s_ref)
  From76/1 -> MATLAB Function2/9(obs_pre)
  From82/1 -> MATLAB Function2/8(target_speed)
  From80/1 -> MATLAB Function2/7(Ego_Ax)
  From79/1 -> MATLAB Function2/6(Ego_Vx)
  From81/1 -> MATLAB Function2/5(Ego_Yaw)
  From78/1 -> MATLAB Function2/4(Ego_y)
  From77/1 -> MATLAB Function2/3(Ego_x)
  MATLAB Function2/1(global_path) -> Goto78/1
  Mux2/1 -> Transpose16/1
  Transpose16/1 -> MATLAB Function9/1(ego_pos)
  Read CM Dict9/1 -> Goto79/1
  From55/1 -> Add/1
  target lane_ Gate/1 -> MATLAB Function2/10(TargetTolgateLane)
  From28/1 -> MATLAB Function5/1(Ego_x)
  From29/1 -> MATLAB Function5/2(Ego_y)
  MATLAB Function5/1(gate_flag) -> Display/1, MATLAB Function11/7(gate_flag), MATLAB Function2/11(gate_flag)
  Transpose23/1 -> MATLAB Function13/1(ego_pos)
  Traffic Object56/1 -> Terminator56/1
  From125/1 -> Transpose19/1
  Bus Selector32/3 -> Mux83/3  "<r_zyx z>"
  Bus Selector44/3 -> Mux108/3  "<r_zyx z>"
  Constant154/1 -> Mux96/2
  Mux81/1 -> Goto93/1
  Bus Selector53/1 -> Mux78/1  "<t_0 x>"
  From138/1 -> MATLAB Function6/1(s_ref)
  From31/1 -> Mux122/12
  From105/1 -> Mux80/2
  Constant188/1 -> Mux119/1
  Traffic Object47/2 -> Bus Selector46/1
  Traffic Object42/2 -> Bus Selector44/1
  From90/1 -> Mux122/21
  From144/1 -> MATLAB Function6/7(Ego_Ax)
  Bus Selector42/1 -> Mux102/1  "<t_0 x>"
  From126/1 -> Mux123/1
  Constant125/1 -> Traffic Object32/1
  Mux98/1 -> Mux97/4
  Read CM Dict16/1 -> Mux115/8
  Constant164/1 -> Mux128/2
  Bus Selector46/5 -> Mux110/5  "<a_0 x>"
  Bus Selector42/6 -> Mux102/6  "<a_0 y>"
  From87/1 -> Mux122/19
  Mux74/1 -> Goto117/1
  Mux84/1 -> Mux83/4
  Traffic Object51/1 -> Terminator51/1
  Bus Selector35/2 -> Mux87/2  "<t_0 y>"
  Bus Selector57/2 -> Mux120/2  "<t_0 y>"
  From92/1 -> Mux122/23
  Constant159/1 -> Mux100/1
  Traffic Object46/2 -> Bus Selector48/1
  Bus Selector45/6 -> Mux106/6  "<a_0 y>"
  Bus Selector34/2 -> Mux85/2  "<t_0 y>"
  Traffic Object36/1 -> Terminator36/1
  Bus Selector35/3 -> Mux87/3  "<r_zyx z>"
  From110/1 -> Mux122/5
  From141/1 -> MATLAB Function6/4(Ego_y)
  Constant170/1 -> Traffic Object45/1
  Mux129/1 -> Goto113/1
  Bus Selector54/7 -> Mux126/7  "<r_zyx z>"
  Bus Selector36/2 -> Mux91/2  "<t_0 y>"
  Constant179/1 -> Goto86/1
  Bus Selector36/1 -> Mux91/1  "<t_0 x>"
  Bus Selector60/3 -> Mux72/3  "<r_zyx z>"
  Bus Selector43/5 -> Mux104/5  "<a_0 x>"
  From109/1 -> Mux122/4
  Mux80/1 -> Transpose23/1
  Traffic Object51/2 -> Bus Selector60/1
  Mux78/1 -> Goto120/1
  From104/1 -> Mux80/1
  Traffic Object36/2 -> Bus Selector35/1
  Read CM Dict19/1 -> Goto80/1
  Constant114/1 -> Mux71/2
  MATLAB Function8/1(lateral_error) -> Goto84/1
  Bus Selector52/2 -> Mux62/2  "<t_0 y>"
  Bus Selector60/2 -> Mux72/2  "<t_0 y>"
  Traffic Object48/1 -> Terminator48/1
  MATLAB Function10/1(poly_coeff) -> Goto83/1
  From99/1 -> Mux122/1
  Read CM Dict20/1 -> Goto81/1
  Bus Selector40/3 -> Mux99/3  "<r_zyx z>"
  Bus Selector57/3 -> Mux120/3  "<r_zyx z>"
  Bus Selector54/5 -> Mux126/5  "<a_0 x>"
  Constant117/1 -> Traffic Object58/1
  Mux105/1 -> Mux104/9
  Mux124/1 -> Goto112/1
  Traffic Object59/1 -> Terminator59/1
  From33/1 -> Mux122/14
  Traffic Object32/2 -> Bus Selector53/1
  Read CM Dict30/1 -> Goto124/1
  Transpose25/1 -> Matrix Concatenate1/2
  Traffic Object55/2 -> Bus Selector52/1
  From108/1 -> Mux122/29
  Bus Selector47/1 -> Mux113/1  "<t_0 x>"
  Constant148/1 -> Traffic Object39/1
  Mux111/1 -> Mux110/9
  Bus Selector45/1 -> Mux106/1  "<t_0 x>"
  Bus Selector52/1 -> Mux62/1  "<t_0 x>"
  Constant145/1 -> Mux92/1
  Bus Selector36/3 -> Mux91/3  "<r_zyx z>"
  From134/1 -> Transpose22/1
  Traffic Object54/1 -> Terminator54/1
  Traffic Object60/1 -> Terminator60/1
  Constant157/1 -> Goto85/1
  Constant193/1 -> Mux125/1
  Constant124/1 -> Mux77/2
  Bus Selector60/1 -> Mux72/1  "<t_0 x>"
  Mux85/1 -> Goto94/1
  Constant136/1 -> Mux86/1
  From119/1 -> MATLAB Function4 1/1(waypoints)
  Bus Selector47/7 -> Mux113/7  "<r_zyx z>"
  Constant153/1 -> Mux96/1
  Bus Selector42/4 -> Mux102/4  "<v_0 y>"
  Mux117/1 -> Goto110/1
  Constant149/1 -> Mux94/1
  Constant195/1 -> Mux125/2
  Transpose21/1 -> Matrix Concatenate1/7
  Constant115/1 -> Traffic Object51/1
  Constant110/1 -> Mux121/1
  Bus Selector38/1 -> Mux93/1  "<t_0 x>"
  Traffic Object46/1 -> Terminator46/1
  Bus Selector49/7 -> Mux115/7  "<r_zyx z>"
  Saturation2/1 -> Write CM Dict2/1, Write CM Dict1/1
  From86/1 -> Mux122/18
  Bus Selector59/2 -> Mux74/2  "<t_0 y>"
  PID Controller3/1 -> Write CM Dict6/1
  Bus Selector39/1 -> Mux95/1  "<t_0 x>"
  Constant182/1 -> Mux114/1
  MATLAB Function6/1(global_path) -> Goto123/1
  Bus Selector59/1 -> Mux74/1  "<t_0 x>"
  Transpose24/1 -> Matrix Concatenate1/1
  Traffic Object35/2 -> Bus Selector34/1
  From111/1 -> Mux122/6
  Traffic Object50/1 -> Terminator50/1
  Traffic Object34/2 -> Bus Selector36/1
  Bus Selector38/2 -> Mux93/2  "<t_0 y>"
  Bus Selector49/4 -> Mux115/4  "<v_0 y>"
  Bus Selector37/1 -> Mux89/1  "<t_0 x>"
  Traffic Object52/2 -> Bus Selector51/1
  Bus Selector39/2 -> Mux95/2  "<t_0 y>"
  Bus Selector56/1 -> Mux129/1  "<t_0 x>"
  Bus Selector47/2 -> Mux113/2  "<t_0 y>"
  Traffic Object58/1 -> Terminator58/1
  Bus Selector40/2 -> Mux99/2  "<t_0 y>"
  Transpose18/1 -> Matrix Concatenate1/4
  Mux99/1 -> Goto101/1
  Traffic Object53/1 -> Terminator53/1
  Mux102/1 -> Goto104/1
  Constant186/1 -> Traffic Object46/1
  Bus Selector45/5 -> Mux106/5  "<a_0 x>"
  Bus Selector51/3 -> Mux124/3  "<r_zyx z>"
  From88/1 -> Mux122/20
  Bus Selector46/1 -> Mux110/1  "<t_0 x>"
  Constant139/1 -> Mux88/1
  Mux72/1 -> Goto118/1
  Constant161/1 -> Mux100/2
  From95/1 -> Mux122/26
  Bus Selector53/2 -> Mux78/2  "<t_0 y>"
  From132/1 -> Transpose21/1
  Traffic Object50/2 -> Bus Selector54/1
  Bus Selector51/1 -> Mux124/1  "<t_0 x>"
  From115/1 -> Mux122/10
  From136/1 -> MATLAB Function12/1(global_waypoint)
  Traffic Object33/2 -> Bus Selector33/1
  Constant197/1 -> Mux127/1
  Bus Selector49/2 -> Mux115/2  "<t_0 y>"
  Bus Selector43/2 -> Mux104/2  "<t_0 y>"
  Constant127/1 -> Mux79/2
  From123/1 -> Transpose17/1
  From133/1 -> Mux7/1
  Mux83/1 -> Goto91/1
  Constant128/1 -> Traffic Object33/1
  Traffic Object45/1 -> Terminator45/1
  Traffic Object34/1 -> Terminator34/1
  Bus Selector33/1 -> Mux81/1  "<t_0 x>"
  Bus Selector54/1 -> Mux126/1  "<t_0 x>"
  Traffic Object58/2 -> Bus Selector59/1
  From117/1 -> Add1/2
  From100/1 -> PID Controller2/1
  Transpose22/1 -> Matrix Concatenate1/8
  From127/1 -> Mux123/2
  Constant146/1 -> Mux90/2
  Traffic Object33/1 -> Terminator33/1
  Mux95/1 -> Goto100/1
  Constant118/1 -> Mux75/1
  Bus Selector45/3 -> Mux106/3  "<v_0 x>"
  Bus Selector43/1 -> Mux104/1  "<t_0 x>"
  Traffic Object55/1 -> Terminator55/1
  From94/1 -> Mux122/25
  Constant113/1 -> Mux71/1
  Mux76/1 -> Goto119/1
  Constant175/1 -> Mux109/2
  Bus Selector46/6 -> Mux110/6  "<a_0 y>"
  Constant144/1 -> Traffic Object34/1
  Bus Selector43/4 -> Mux104/4  "<v_0 y>"
  From114/1 -> Mux122/9
  Constant129/1 -> Mux82/1
  Bus Selector42/7 -> Mux102/7  "<r_zyx z>"
  Read CM Dict11/1 -> Mux104/8
  Mux101/1 -> Mux62/4
  Mux107/1 -> Mux106/9
  From112/1 -> Mux122/7
  Traffic Object57/2 -> Bus Selector56/1
  Constant160/1 -> Mux98/2
  Traffic Object40/2 -> Bus Selector39/1
  Mux87/1 -> Goto95/1
  Traffic Object41/1 -> Terminator41/1
  Constant174/1 -> Mux107/2
  Bus Selector59/3 -> Mux74/3  "<r_zyx z>"
  Traffic Object47/1 -> Terminator47/1
  Bus Selector42/5 -> Mux102/5  "<a_0 x>"
  Mux73/1 -> Mux72/4
  Traffic Object60/2 -> Bus Selector58/1
  MATLAB Function1/1(target_speed) -> Rate Limiter1/1
  Mux126/1 -> Goto114/1
  Bus Selector37/3 -> Mux89/3  "<r_zyx z>"
  MATLAB Function13/1(ego_lane_idx) -> Goto90/1
  Bus Selector49/3 -> Mux115/3  "<v_0 x>"
  Traffic Object52/1 -> Terminator52/1
  Constant180/1 -> Mux111/2
  Bus Selector42/3 -> Mux102/3  "<v_0 x>"
  Bus Selector48/5 -> Mux117/5  "<a_0 x>"
  Bus Selector46/2 -> Mux110/2  "<t_0 y>"
  Constant177/1 -> Traffic Object47/1
  Mux71/1 -> Mux70/4
  From147/1 -> MATLAB Function10/1(local_waypoints)
  Bus Selector43/3 -> Mux104/3  "<v_0 x>"
  Constant131/1 -> Traffic Object53/1
  Traffic Object44/2 -> Bus Selector43/1
  From143/1 -> Mux7/2
  From142/1 -> MATLAB Function6/6(Ego_Vx)
  From113/1 -> Mux122/8
  Traffic Object59/2 -> Bus Selector57/1
  Gain1/1 -> Saturation2/1
  Constant151/1 -> Traffic Object40/1
  Constant137/1 -> Mux86/2
  PID Controller2/1 -> Gain1/1
  From91/1 -> Mux122/22
  Transpose17/1 -> Matrix Concatenate1/3
  Read CM Dict13/1 -> Mux117/8
  Bus Selector42/2 -> Mux102/2  "<t_0 y>"
  Bus Selector48/2 -> Mux117/2  "<t_0 y>"
  Bus Selector41/1 -> Mux97/1  "<t_0 x>"
  Matrix Concatenate1/1 -> Goto97/1
  Mux82/1 -> Mux81/4
  Constant181/1 -> Traffic Object48/1
  Constant165/1 -> Mux103/2
  From107/1 -> Mux122/2
  Constant134/1 -> Mux84/2
  Constant185/1 -> Mux116/1
  Bus Selector54/2 -> Mux126/2  "<t_0 y>"
  From93/1 -> Mux122/24
  Mux115/1 -> Goto111/1
  Constant143/1 -> Mux90/1
  Traffic Object38/1 -> Terminator38/1
  Constant138/1 -> Traffic Object36/1
  Bus Selector48/1 -> Mux117/1  "<t_0 x>"
  Bus Selector54/3 -> Mux126/3  "<v_0 x>"
  Bus Selector57/1 -> Mux120/1  "<t_0 x>"
  Traffic Object35/1 -> Terminator35/1
  Bus Selector50/2 -> Mux76/2  "<t_0 y>"
  Bus Selector43/7 -> Mux104/7  "<r_zyx z>"
  From140/1 -> MATLAB Function6/3(Ego_x)
  MATLAB Function4 1/1(local_waypoints_) -> Goto75/1
  Bus Selector47/6 -> Mux113/6  "<a_0 y>"
  From85/1 -> Mux122/17
  Bus Selector49/5 -> Mux115/5  "<a_0 x>"
  From139/1 -> MATLAB Function6/9(obs_pre)
  Constant162/1 -> Traffic Object43/1
  Mux125/1 -> Mux124/4
  From129/1 -> MATLAB Function1/4(ego_lane_idx)
  From89/1 -> Mux122/3
  From102/1 -> MATLAB Function13/4(wp2)
  Read CM Dict12/1 -> Mux106/8
  Traffic Object45/2 -> Bus Selector45/1
  Bus Selector49/1 -> Mux115/1  "<t_0 x>"
  Mux118/1 -> Mux117/9
  Constant187/1 -> Mux118/1
  Mux120/1 -> Goto115/1
  Traffic Object37/1 -> Terminator37/1
  MATLAB Function13/2(traffic_lane_idx) -> Goto89/1
  From145/1 -> MATLAB Function6/5(Ego_Yaw)
  Bus Selector58/2 -> Mux70/2  "<t_0 y>"
  Bus Selector46/4 -> Mux110/4  "<v_0 y>"
  Traffic Object39/2 -> Bus Selector38/1
  Constant189/1 -> Mux116/2
  From120/1 -> Transpose24/1
  Constant167/1 -> Mux105/1
  Bus Selector37/2 -> Mux89/2  "<t_0 y>"
  Bus Selector45/2 -> Mux106/2  "<t_0 y>"
  Bus Selector39/3 -> Mux95/3  "<r_zyx z>"
  Read CM Dict14/1 -> Mux110/8
  Constant150/1 -> Mux94/2
  Constant133/1 -> Mux82/2
  Bus Selector55/3 -> Mux112/3  "<r_zyx z>"
  Constant141/1 -> Traffic Object56/1
  Constant122/1 -> Traffic Object54/1
  Constant169/1 -> Mux105/2
  Bus Selector50/1 -> Mux76/1  "<t_0 x>"
  Mux100/1 -> Mux99/4
  From106/1 -> Mux122/28
  From118/1 -> Add1/1
  Read CM Dict18/1 -> Goto77/1
  Mux93/1 -> Goto99/1
  Constant132/1 -> Mux84/1
  Bus Selector55/2 -> Mux112/2  "<t_0 y>"
  Bus Selector32/1 -> Mux83/1  "<t_0 x>"
  Constant158/1 -> Traffic Object38/1
  From83/1 -> Mux122/15
  Traffic Object43/2 -> Bus Selector42/1
  Traffic Object49/1 -> Terminator49/1
  Mux79/1 -> Mux78/4
  From98/1 -> MATLAB Function8/2(velocity)
  Traffic Object39/1 -> Terminator39/1
  Mux116/1 -> Mux115/9
  From32/1 -> Mux122/13
  Constant147/1 -> Mux92/2
  Read CM Dict10/1 -> Mux102/8
  Constant108/1 -> Traffic Object55/1
  Constant190/1 -> Goto87/1
  Bus Selector33/3 -> Mux81/3  "<r_zyx z>"
  From135/1 -> MATLAB Function1/3(ego_vx)
  Mux91/1 -> Goto96/1
  Constant196/1 -> Traffic Object50/1
  From116/1 -> MATLAB Function1/5(traffic_info), MATLAB Function13/2(traffic_info)
  Read CM Dict17/1 -> Mux126/8
  Bus Selector43/6 -> Mux104/6  "<a_0 y>"
  MATLAB Function1/2(debug_time_gap) -> Scope1/1
  Constant107/1 -> Goto121/1
  Mux121/1 -> Mux120/4
  Bus Selector50/3 -> Mux76/3  "<r_zyx z>"
  Bus Selector54/4 -> Mux126/4  "<v_0 y>"
  Bus Selector58/1 -> Mux70/1  "<t_0 x>"
  Read CM Dict15/1 -> Mux113/8
  Constant173/1 -> Mux109/1
  From137/1 -> MATLAB Function6/2(global_waypoint_2)
  Constant111/1 -> Mux121/2
  Constant116/1 -> Mux73/1
  Add1/1 -> PID Controller3/1
  Constant120/1 -> Mux73/2
  Mux113/1 -> Goto109/1
  Transpose19/1 -> Matrix Concatenate1/5
  Rate Limiter1/1 -> Goto92/1
  Bus Selector41/2 -> Mux97/2  "<t_0 y>"
  Constant155/1 -> Traffic Object41/1
  Mux119/1 -> Mux129/4
  Constant135/1 -> Traffic Object35/1
  From131/1 -> Transpose20/1
  Constant163/1 -> Mux103/1
  From103/1 -> MATLAB Function13/5(wp3)
  Constant112/1 -> Traffic Object60/1
  Mux104/1 -> Goto105/1
  Mux114/1 -> Mux113/9
  Constant178/1 -> Mux111/1
  Traffic Object40/1 -> Terminator40/1
  Constant172/1 -> Traffic Object42/1
  Constant156/1 -> Mux98/1
  Constant198/1 -> Mux127/2
  Traffic Object48/2 -> Bus Selector47/1
  Bus Selector33/2 -> Mux81/2  "<t_0 y>"
  From122/1 -> MATLAB Function4 1/3(head)
  Bus Selector48/3 -> Mux117/3  "<v_0 x>"
  Constant152/1 -> Mux128/1
  MATLAB Function12/1(s_ref) -> Goto122/1
  Constant130/1 -> Mux101/2
  Bus Selector54/6 -> Mux126/6  "<a_0 y>"
  Mux88/1 -> Mux87/4
  Mux109/1 -> Mux108/4
  Mux90/1 -> Mux89/4
  Mux7/1 -> MATLAB Function4 1/2(vehicle_position)
  Constant171/1 -> Mux107/1
  Traffic Object53/2 -> Bus Selector32/1
  Constant121/1 -> Mux75/2
  Bus Selector51/2 -> Mux124/2  "<t_0 y>"
  Constant194/1 -> Mux119/2
  Traffic Object32/1 -> Terminator32/1
  From130/1 -> MATLAB Function1/6(traffic_lane_idx)
  Bus Selector32/2 -> Mux83/2  "<t_0 y>"
  Traffic Object37/2 -> Bus Selector37/1
  Bus Selector47/4 -> Mux113/4  "<v_0 y>"
  Bus Selector34/3 -> Mux85/3  "<r_zyx z>"
  Bus Selector38/3 -> Mux93/3  "<r_zyx z>"
  Constant183/1 -> Mux114/2
  Traffic Object57/1 -> Terminator57/1
  Mux112/1 -> Goto103/1
  Constant109/1 -> Traffic Object59/1
  Bus Selector48/7 -> Mux117/7  "<r_zyx z>"
  Constant142/1 -> Traffic Object37/1
  Bus Selector47/3 -> Mux113/3  "<v_0 x>"
  Constant176/1 -> Traffic Object57/1
  Bus Selector47/5 -> Mux113/5  "<a_0 x>"
  Traffic Object54/2 -> Bus Selector50/1
  From97/1 -> MATLAB Function8/1(poly_coeff)
  Transpose20/1 -> Matrix Concatenate1/6
  Traffic Object49/2 -> Bus Selector49/1
  Bus Selector56/3 -> Mux129/3  "<r_zyx z>"
  From121/1 -> Transpose25/1
  Constant126/1 -> Mux79/1
  Mux89/1 -> Goto98/1
  Traffic Object44/1 -> Terminator44/1
  Constant166/1 -> Traffic Object44/1
  Constant168/1 -> MATLAB Function8/3(lookahead_time)
  From30/1 -> Mux122/11
  Constant140/1 -> Mux88/2
  Traffic Object38/2 -> Bus Selector40/1
  Traffic Object56/2 -> Bus Selector55/1
  From84/1 -> Mux122/16
  Traffic Object41/2 -> Bus Selector41/1
  Mux128/1 -> Mux112/4
  Constant191/1 -> Mux118/2
  Constant184/1 -> Traffic Object49/1
  Read CM Dict21/1 -> Goto82/1
  Bus Selector48/6 -> Mux117/6  "<a_0 y>"
  From101/1 -> MATLAB Function13/3(wp1)
  Constant119/1 -> Mux101/1
  Bus Selector49/6 -> Mux115/6  "<a_0 y>"
  Bus Selector46/3 -> Mux110/3  "<v_0 x>"
  Mux122/1 -> Traffic_Info1/1
  From124/1 -> Transpose18/1
  Mux127/1 -> Mux126/9
  Bus Selector46/7 -> Mux110/7  "<r_zyx z>"
  Mux123/1 -> MATLAB Function1/1(ego_pos)
  Mux70/1 -> Goto116/1
  From96/1 -> Mux122/27
  Bus Selector58/3 -> Mux70/3  "<r_zyx z>"
  Bus Selector41/3 -> Mux97/3  "<r_zyx z>"
  Mux108/1 -> Goto106/1
  Mux92/1 -> Mux91/4
  Constant192/1 -> Traffic Object52/1
  Mux75/1 -> Mux74/4
  Bus Selector40/1 -> Mux99/1  "<t_0 x>"
  Mux106/1 -> Goto107/1
  Bus Selector45/7 -> Mux106/7  "<r_zyx z>"
  From146/1 -> MATLAB Function6/8(target_speed)
  Mux86/1 -> Mux85/4
  Bus Selector34/1 -> Mux85/1  "<t_0 x>"
  Mux62/1 -> Goto88/1
  Bus Selector55/1 -> Mux112/1  "<t_0 x>"
  Bus Selector35/1 -> Mux87/1  "<t_0 x>"
  Traffic Object43/1 -> Terminator43/1
  Bus Selector52/3 -> Mux62/3  "<r_zyx z>"
  Mux96/1 -> Mux95/4
  Bus Selector45/4 -> Mux106/4  "<v_0 y>"
  Traffic Object42/1 -> Terminator42/1
  Bus Selector53/3 -> Mux78/3  "<r_zyx z>"
  Bus Selector44/1 -> Mux108/1  "<t_0 x>"
  Mux103/1 -> Mux102/9
  Constant123/1 -> Mux77/1
  Mux110/1 -> Goto108/1
  Mux94/1 -> Mux93/4
  Bus Selector48/4 -> Mux117/4  "<v_0 y>"
  Bus Selector44/2 -> Mux108/2  "<t_0 y>"
  From128/1 -> MATLAB Function1/2(ego_yaw)
  Bus Selector56/2 -> Mux129/2  "<t_0 y>"
  Mux77/1 -> Mux76/4
  Mux97/1 -> Goto102/1
  MATLAB Function/2(en_Go2Park) -> [Enable_Go2Park]
  Matrix Concatenate3/1 -> [route_waypoint]
  Chart/1(do_Logic()) -> Function-Call Split/1
  Constant201/1 -> Pad2/1
  Function-Call Split/1 -> Goto125/1
  Function-Call Split/2 -> Goto126/1
  Constant200/1 -> Pad1/1
  Enabled Subsystem1/2(Output1) -> Scope4/1, MATLAB Function/2(Go2Park_finish_flag)
  [Enable_Parking] -> Unit Delay2/1
  Read CM Dict31/1 -> MATLAB Function14/1(Ego_x)
  Constant199/1 -> Pad/1
  Pad2/1 -> Matrix Concatenate3/3
  Read CM Dict32/1 -> MATLAB Function14/2(Ego_y)
  Unit Delay/1 -> Enabled Subsystem/Enable
  MATLAB Function/3(en_Parking) -> [Enable_Parking]
  [Enable_Go2Park] -> Unit Delay1/1
  MATLAB Function/1(en_Driving) -> [Enable_Driving]
  Unit Delay2/1 -> Enabled Subsystem2/Enable, Scope3/1
  [route_waypoint] -> MATLAB Function14/3(waypoint)
  Unit Delay1/1 -> Enabled Subsystem1/Enable
  [Enable_Driving] -> Unit Delay/1
  Pad1/1 -> Matrix Concatenate3/2
  Pad/1 -> Matrix Concatenate3/1
  MATLAB Function14/1(Driving_finish_flag) -> MATLAB Function/1(Driving_finish_flag)
  MATLAB Function19/1(gate_flag) -> MATLAB Function16/11(gate_flag), MATLAB Function15/7(gate_flag), Display1/1
  From153/1 -> MATLAB Function19/2(Ego_y)
  From152/1 -> MATLAB Function19/1(Ego_x)
  target lane_ Gate1/1 -> MATLAB Function16/10(TargetTolgateLane)
  From158/1 -> Add2/1
  MATLAB Function16/1(global_path) -> Goto135/1
  From166/1 -> MATLAB Function16/3(Ego_x)
  From167/1 -> MATLAB Function16/4(Ego_y)
  From171/1 -> MATLAB Function16/5(Ego_Yaw)
  From168/1 -> MATLAB Function16/6(Ego_Vx)
  From170/1 -> MATLAB Function16/7(Ego_Ax)
  From172/1 -> MATLAB Function16/8(target_speed)
  From165/1 -> MATLAB Function16/9(obs_pre)
  From164/1 -> MATLAB Function16/1(s_ref)
  From163/1 -> MATLAB Function16/2(global_waypoint_2)
  MATLAB Function20/1(s_ref) -> Goto134/1
  From173/1 -> PID Controller4/1
  From161/1 -> MATLAB Function15/6(traffic_lane_idx)
  MATLAB Function15/2(debug_time_gap) -> ?
  PID Controller4/1 -> Gain2/1
  MATLAB Function4 2/1(local_waypoints_) -> Goto131/1, To Workspace3/1
  Saturation3/1 -> Write CM Dict7/1, Write CM Dict8/1
  MATLAB Function17/1(lateral_error) -> Goto133/1
  Mux130/1 -> MATLAB Function4 2/2(vehicle_position)
  From169/1 -> MATLAB Function17/2(velocity)
  From155/1 -> Mux130/1
  From160/1 -> MATLAB Function18/1(local_waypoints)
  Constant202/1 -> MATLAB Function17/3(lookahead_time)
  MATLAB Function18/1(poly_coeff) -> Scope5/1, Goto132/1
  From159/1 -> MATLAB Function4 2/1(waypoints), To Workspace2/1
  Gain2/1 -> Saturation3/1
  From162/1 -> MATLAB Function17/1(poly_coeff)
  PID Controller5/1 -> Write CM Dict9/1
  From154/1 -> MATLAB Function4 2/3(head)
  Add2/1 -> PID Controller5/1
  From157/1 -> Add2/2
  From156/1 -> Mux130/2
